simulink library "dinr"  (Simulink 8.2)
settings: Solver=ode45  SolverMode=SingleTasking  StartTime=0.0  StopTime=10.0  RelTol=1e-3
undefined symbols (not defined in the file or in its folder): FALSE, KDINR_DisableEstimator_flg, TRUE
libraries: simulink x2
(part 2 of 2)

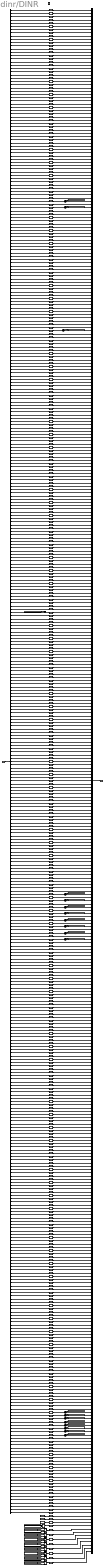
== system dinr/DINR ==
  BINP_outputs : Inport  OutDataTypeStr=Bus: BINP_outputs
  trig_DINR : TriggerPort  TriggerType=function-call
  Bus Selector : BusSelector  OutputSignals=VINP_IgnitionVolt_V,VINP_IgnitionVoltValid_flg,VINP_BatteryVolt_V,VINP_BatteryVoltValid_flg,VINP_AppTime_ms,VINP_ADCFault_enum,VINP_EEPROMFault_enum,VINP_RAMFault_enum,VINP_ROMFault_enum,VINP_VREF1Fault_enum,VINP_VREF2Fault_enum,VINP_AccelPedalPosn_pct,VINP_AccelPedalPosnValid_flg,VINP_EffAccelPedalPosn_pct,VINP_EffAccelPedalPosnValid_flg,VINP_EngSpd_erpm,VINP_EngSpdValid_flg,VINP_EngTqFriction_Nm,VINP_EngTqFrictionValid_flg,VINP_EngTqIndicated_Nm,VINP_EngTqIndicatedValid_flg,VINP_EngTqIndicatedCOR_Nm,VINP_EngTqIndicatedCORValid_flg,VINP_EngTqMax_Nm,VINP_EngTqMaxValid_flg,VINP_EngTqMin_Nm,VINP_EngTqMinValid_flg,VINP_EngTqUnCORFault_flg,VINP_EngTqUnCORFaultValid_flg,VINP_EMSHybridOpState_enum,VINP_EMSHybridOpStateValid_flg,VINP_EMSOpState_enum,VINP_EMSOpStateValid_flg,VINP_EngHoodOpen_flg,VINP_EngHoodOpenValid_flg,VINP_OBDWarnCycAchiv_flg,VINP_OBDWarnCycAchivValid_flg,VINP_OBDDriveCycAchiv_flg,VINP_OBDDriveCycAchivValid_flg,VINP_ShifterPosn_enum,VINP_ShifterPosnValid_flg,VINP_NowGearPosn_enum,VINP_NowGearPosnValid_flg,VINP_TMTurbineSpd_rpm,VINP_TMTurbineSpdValid_flg,VINP_TCMFaultStatus_enum,VINP_TCMFaultStatusValid_flg,VINP_TqConvClutchSt_enum,VINP_TqConvClutchStValid_flg,VINP_TCMMILReq_flg,VINP_TCMMILReqValid_flg,VINP_TCMWinterMode_flg,VINP_TCMWinterModeValid_flg,VINP_TCMPowerMode_flg,VINP_TCMPowerModeValid_flg,VINP_DriverMode_enum,VINP_DriverModeValid_flg,VINP_KeySwitchStatus_enum,VINP_KeySwitchStatusValid_flg,VINP_TurnSignalSwL_flg,VINP_TurnSignalSwLValid_flg,VINP_TurnSignalSwR_flg,VINP_TurnSignalSwRValid_flg,VINP_HazardLightSw_flg,VINP_HazardLightSwValid_flg,VINP_DriverDoorOpen_flg,VINP_DriverDoorOpenValid_flg,VINP_PassengerDoorOpen_flg,VINP_PassengerDoorOpenValid_flg,VINP_LRDoorOpen_flg,VINP_LRDoorOpenValid_flg,VINP_RRDoorOpen_flg,VINP_RRDoorOpenValid_flg,VINP_TailGateOpen_flg,VINP_TailGateOpenValid_flg,VINP_AnyDoorOpen_flg,VINP_AnyDoorOpenValid_flg,VINP_VehCrashed_flg,VINP_VehCrashedValid_flg,VINP_ABSActive_flg,VINP_ABSActiveValid_flg,VINP_ABSFault_flg,VINP_ABSFaultValid_flg,VINP_EBDFault_flg,VINP_EBDFaultValid_flg,VINP_ESCActive_flg,VINP_ESCActiveValid_flg,VINP_ESCFault_flg,VINP_ESCFaultValid_flg,VINP_TCSActive_flg,VINP_TCSActiveValid_flg,VINP_TCSEnabled_flg,VINP_TCSEnabledValid_flg,VINP_TCSFault_flg,VINP_TCSFaultValid_flg,VINP_HSAActive_flg,VINP_HSAActiveValid_flg,VINP_HSAFault_flg,VINP_HSAFaultValid_flg,VINP_BrkLampOn_flg,VINP_BrkLampOnValid_flg,VINP_VehSpd_kph,VINP_VehSpdValid_flg,VINP_YawRate_degps,VINP_YawRateValid_flg,VINP_LatAccel_G,VINP_LatAccelValid_flg,VINP_LongAccel_G,VINP_LongAccelValid_flg,VINP_MCPressure_bar,VINP_MCPressureValid_flg,VINP_SurfaceGrade_deg,VINP_SurfaceGradeValid_flg,VINP_BrakBoosterPres_kPa,VINP_BrakBoosterPresValid_flg,VINP_LowBrakBoosterPres_flg,VINP_LowBrakBoosterPresValid_flg,VINP_LFWheelSpeed_kph,VINP_LFWheelSpeedValid_flg,VINP_LRWheelSpeed_kph,VINP_LRWheelSpeedValid_flg,VINP_RFWheelSpeed_kph,VINP_RFWheelSpeedValid_flg,VINP_RRWheelSpeed_kph,VINP_RRWheelSpeedValid_flg,VINP_SteerAngle_deg,VINP_SteerAngleValid_flg,VINP_SteerSpeed_degps,VINP_SteerSpeedValid_flg,VINP_RelSteerAngle_deg,VINP_RelSteerAngleValid_flg,VINP_SteerTorque_Nm,VINP_SteerTorqueValid_flg,VINP_EPSElectPWR_A,VINP_EPSElectPWRValid_flg,VINP_EPSFailed_flg,VINP_EPSFailedValid_flg,VINP_AckCurStrAngReq_deg,VINP_AckCurStrAngReqValid_flg,VINP_AckCurStrAngReqApplable_flg,VINP_AckCurStrAngReqApplableValid_flg,VINP_AckCurStrTqReq_Nm,VINP_AckCurStrTqReqValid_flg,VINP_AckCurStrTqReqApplable_flg,VINP_AckCurStrTqReqApplableValid_flg,VINP_EPSBattVolt_V,VINP_EPSBattVoltValid_flg,VINP_EPASMILReq_flg,VINP_EPASMILReqValid_flg,VINP_EPSLKAStatus_enum,VINP_EPSLKAStatusValid_flg,VINP_EPSLFCStatus_enum,VINP_EPSLFCStatusValid_flg,VINP_EPSADASAbReason_enum,VINP_EPSADASAbReasonValid_flg,VINP_OdoMeter_km,VINP_OdoMeterValid_flg,VINP_LowBrakeFluid_flg,VINP_LowBrakeFluidValid_flg,VINP_ParkBrakeOn_flg,VINP_ParkBrakeOnValid_flg,VINP_SeatBeltNOTFasten_flg,VINP_SeatBeltNOTFastenValid_flg,VINP_MeterVehSpd_kph,VINP_MeterVehSpdValid_flg,VINP_OutsideTemp_degC,VINP_OutsideTempValid_flg,VINP_ParkBrakeBindSta_enum,VINP_ParkBrakeBindStaValid_flg,VINP_RearFogSwOn_flg,VINP_RearFogSwOnValid_flg,VINP_HighBeamSwOn_flg,VINP_HighBeamSwOnValid_flg,VINP_AckCurBrakDecReq_mps2,VINP_AckCurBrakDecReqValid_flg,VINP_AckCurBrakDecReqApplable_flg,VINP_AckCurBrakDecReqApplableValid_flg,VINP_AckCurPTTqReq_Nm,VINP_AckCurPTTqReqValid_flg,VINP_AckCurPTTqReqApplable_flg,VINP_AckCurPTTqReqApplableValid_flg,VINP_AckCurVehDec_mps2,VINP_AckCurVehDecValid_flg,VINP_DeceContManag_flg,VINP_DeceContManagValid_flg,VINP_DriverBrakPedalOn_flg,VINP_DriverBrakPedalOnValid_flg,VINP_ECMExtnTqAvailable_flg,VINP_ECMExtnTqAvailableValid_flg,VINP_ECMTqSource_enum,VINP_ECMTqSourceValid_flg,VINP_ESCBrakeStatus_enum,VINP_ESCBrakeStatusValid_flg,VINP_ESCExtnBrkAvailable_flg,VINP_ESCExtnBrkAvailableValid_flg,VINP_ESCBattVolt_V,VINP_ESCBattVoltValid_flg,VINP_HWAccelPedalPosn_pct,VINP_HWAccelPedalPosnValid_flg,VINP_CurDriverTqReq_Nm,VINP_CurDriverTqReqValid_flg,VINP_TCMGearPosnReqAllow_enum,VINP_TCMGearPosnReqAllowValid_flg,VINP_MSAStatus_enum,VINP_MSAStatusValid_flg,VINP_HybridLimpHome_flg,VINP_HybridLimpHomeValid_flg,VINP_HCUMILReq_flg,VINP_HCUMILReqValid_flg,VINP_ACCOnVCU_flg,VINP_ACCOnVCUValid_flg,VINP_ACCResSpdIncVCU_flg,VINP_ACCResSpdIncVCUValid_flg,VINP_ACCSetSpdDecVCU_flg,VINP_ACCSetSpdDecVCUValid_flg,VINP_ACCDistVCU_flg,VINP_ACCDistVCUValid_flg,VINP_ACCTimeGapIncVCU_flg,VINP_ACCTimeGapIncVCUValid_flg,VINP_ACCTimeGapDecVCU_flg,VINP_ACCTimeGapDecVCUValid_flg,VINP_LFCOnVCU_flg,VINP_LFCOnVCUValid_flg,VINP_MSAOnVCU_flg,VINP_MSAOnVCUValid_flg,VINP_AEBEnableH_flg,VINP_AEBEnableHValid_flg,VINP_FCWEnableH_flg,VINP_FCWEnableHValid_flg,VINP_CSCEnableH_flg,VINP_CSCEnableHValid_flg,VINP_LKAEnableH_flg,VINP_LKAEnableHValid_flg,VINP_MAPAEnableH_flg,VINP_MAPAEnableHValid_flg,VINP_LCSEnableH_flg,VINP_LCSEnableHValid_flg,VINP_FCWWarningModeH_enum,VINP_FCWWarningModeHValid_flg,VINP_DefMaxACCSetSpeed_kph,VINP_DefMaxACCSetSpeedValid_flg,VINP_LFCPilotOnH_flg,VINP_LFCPilotOnHValid_flg,VINP_LFCPilotCancelH_flg,VINP_LFCPilotCancelHValid_flg,VINP_ACCOnH_flg,VINP_ACCOnHValid_flg,VINP_ACCCancelH_flg,VINP_ACCCancelHValid_flg,VINP_ACCResSpdIncH_flg,VINP_ACCResSpdIncHValid_flg,VINP_ACCSetSpdDecH_flg,VINP_ACCSetSpdDecHValid_flg,VINP_ACCSpdIncH_flg,VINP_ACCSpdIncHValid_flg,VINP_ACCSpdDecH_flg,VINP_ACCSpdDecHValid_flg,VINP_ACCTimeGapIncH_flg,VINP_ACCTimeGapIncHValid_flg,VINP_ACCTimeGapDecH_flg,VINP_ACCTimeGapDecHValid_flg,VINP_IGSAOnH_flg,VINP_IGSAOnHValid_flg,VINP_IGSAResSpdIncH_flg,VINP_IGSAResSpdIncHValid_flg,VINP_IGSASetSpdDecH_flg,VINP_IGSASetSpdDecHValid_flg,VINP_IGSASwitchModeH_flg,VINP_IGSASwitchModeHValid_flg,VINP_LaneQualityL_enum,VINP_LaneQualityLValid_flg,VINP_LaneQualityR_enum,VINP_LaneQualityRValid_flg,VINP_LaneC0LRaw_m,VINP_LaneC0LValid_flg,VINP_LaneC1LRaw_rad,VINP_LaneC1LValid_flg,VINP_LaneC2LRaw_rat,VINP_LaneC2LValid_flg,VINP_LaneC3LRaw_rat,VINP_LaneC3LValid_flg,VINP_LaneC0RRaw_m,VINP_LaneC0RValid_flg,VINP_LaneC1RRaw_rad,VINP_LaneC1RValid_flg,VINP_LaneC2RRaw_rat,VINP_LaneC2RValid_flg,VINP_LaneC3RRaw_rat,VINP_LaneC3RValid_flg,VINP_LaneTypeL_enum,VINP_LaneTypeLValid_flg,VINP_LaneTypeR_enum,VINP_LaneTypeRValid_flg,VINP_LaneMrkClrL_enum,VINP_LaneMrkClrLValid_flg,VINP_LaneMrkClrR_enum,VINP_LaneMrkClrRValid_flg,VINP_LaneMrkWidL_m,VINP_LaneMrkWidLValid_flg,VINP_LaneMrkWidR_m,VINP_LaneMrkWidRValid_flg,VINP_ViewRangeStartL_m,VINP_ViewRangeStartLValid_flg,VINP_ViewRangeStartR_m,VINP_ViewRangeStartRValid_flg,VINP_ViewRangeEndL_m,VINP_ViewRangeEndLValid_flg,VINP_ViewRangeEndR_m,VINP_ViewRangeEndRValid_flg,VINP_TLCL_s,VINP_TLCLValid_flg,VINP_TLCR_s,VINP_TLCRValid_flg,VINP_LaneCrosL_flg,VINP_LaneCrosLValid_flg,VINP_LaneCrosR_flg,VINP_LaneCrosRValid_flg,VINP_NextLaneC0L_m,VINP_NextLaneC0LValid_flg,VINP_NextLaneC1L_rad,VINP_NextLaneC1LValid_flg,VINP_NextLaneC2L_rat,VINP_NextLaneC2LValid_flg,VINP_NextLaneC3L_rat,VINP_NextLaneC3LValid_flg,VINP_NextLaneQualityL_enum,VINP_NextLaneQualityLValid_flg,VINP_NextLaneTypeL_enum,VINP_NextLaneTypeLValid_flg,VINP_NextLaneMrkWidL_m,VINP_NextLaneMrkWidLValid_flg,VINP_NextViewRangeStartL_m,VINP_NextViewRangeStartLValid_flg,VINP_NextViewRangeEndL_m,VINP_NextViewRangeEndLValid_flg,VINP_NextLaneC0R_m,VINP_NextLaneC0RValid_flg,VINP_NextLaneC1R_rad,VINP_NextLaneC1RValid_flg,VINP_NextLaneC2R_rat,VINP_NextLaneC2RValid_flg,VINP_NextLaneC3R_rat,VINP_NextLaneC3RValid_flg,VINP_NextLaneQualityR_enum,VINP_NextLaneQualityRValid_flg,VINP_NextLaneTypeR_enum,VINP_NextLaneTypeRValid_flg,VINP_NextLaneMrkWidR_m,VINP_NextLaneMrkWidRValid_flg,VINP_NextViewRangeStartR_m,VINP_NextViewRangeStartRValid_flg,VINP_NextViewRangeEndR_m,VINP_NextViewRangeEndRValid_flg,VINP_CamNofObjects_num,VINP_CamNofObjectsValid_flg,VINP_CamGoDecision_enum,VINP_CamGoDecisionValid_flg,VINP_CloseCarDetected_flg,VINP_CloseCarDetectedValid_flg,VINP_RightCarCutIn_flg,VINP_RightCarCutInValid_flg,VINP_LeftCarCutIn_flg,VINP_LeftCarCutInValid_flg,VINP_CamFSImpairedVD_flg,VINP_CamFSImpairedVDValid_flg,VINP_CamFSLowSun_flg,VINP_CamFSLowSunValid_flg,VINP_CamFSBlurImage_flg,VINP_CamFSBlurImageValid_flg,VINP_CamFSSmearImage_flg,VINP_CamFSSmearImageValid_flg,VINP_CamFSPartialBlockage_flg,VINP_CamFSPartialBlockageValid_flg,VINP_CamFSFullBlockage_flg,VINP_CamFSFullBlockageValid_flg,VINP_CamFSSplashes_flg,VINP_CamFSSplashesValid_flg,VINP_CamFSOutofCal_flg,VINP_CamFSOutofCalValid_flg,VINP_CamFSCalMisalign_flg,VINP_CamFSCalMisalignValid_flg,VINP_CamFSSmearedspots_flg,VINP_CamFSSmearedspotsValid_flg,VINP_CamFSSpotHalosFrozen_flg,VINP_CamFSSpotHalosFrozenValid_flg,VINP_CamFSFoggySpots_flg,VINP_CamFSFoggySpotsValid_flg,VINP_CamFSSunRay_flg,VINP_CamFSSunRayValid_flg,VINP_CamObsID10_num,VINP_CamObsIDValid10_flg,VINP_CamObsPosX10_m,VINP_CamObsPosXValid10_flg,VINP_CamObsPosY10_m,VINP_CamObsPosYValid10_flg,VINP_CamObsVelX10_mps,VINP_CamObsVelXValid10_flg,VINP_CamObsVelY10_mps,VINP_CamObsVelYValid10_flg,VINP_CamObsAccX10_mps2,VINP_CamObsAccXValid10_flg,VINP_CamObsAng10_deg,VINP_CamObsAngValid10_flg,VINP_CamObsAngRate10_degps,VINP_CamObsAngRateValid10_flg,VINP_CamObsLength10_m,VINP_CamObsLengthValid10_flg,VINP_CamObsWidth10_m,VINP_CamObsWidthValid10_flg,VINP_CamObsType10_enum,VINP_CamObsTypeValid10_flg,VINP_CamObsStatus10_enum,VINP_CamObsStatusValid10_flg,VINP_CamObsValid10_enum,VINP_CamObsValidValid10_flg,VINP_CamObsMoveInO10_enum,VINP_CamObsMoveInOValid10_flg,VINP_CamObsBlinker10_enum,VINP_CamObsBlinkerValid10_flg,VINP_CamObsBrakeLight10_flg,VINP_CamObsBrakeLightValid10_flg,VINP_CamObsAge10_cnt,VINP_CamObsAgeValid10_flg,VINP_CamObsLane10_enum,VINP_CamObsLaneValid10_flg,VINP_CamObsCIPV10_flg,VINP_CamObsCIPVValid10_flg,VINP_CamObsReplaced10_flg,VINP_CamObsReplacedValid10_flg,VINP_IgnitionActive_flg,VINP_VehSpd_mps,VINP_SteerAngle_rad,VINP_YawRate_radps,VINP_LaneC0LKalF_m,VINP_LaneC1LKalF_rad,VINP_LaneC2LKalF_rat,VINP_LaneC3LKalF_rat,VINP_LaneC0RKalF_m,VINP_LaneC1RKalF_rad,VINP_LaneC2RKalF_rat,VINP_LaneC3RKalF_rat,VINP_ABSCANValid_flg,VINP_BCMCANValid_flg,VINP_ECMCANValid_flg,VINP_TCMCANValid_flg,VINP_EPSCANValid_flg,VINP_METERCANValid_flg,VINP_ACCANValid_flg,VINP_EPBCANValid_flg,VINP_VCUCANValid_flg,VINP_HMICANValid_flg,VINP_CSWCANValid_flg,VINP_EPMCANValid_flg,VINP_ABSCANAlive_flg,VINP_BCMCANAlive_flg,VINP_ECMCANAlive_flg,VINP_TCMCANAlive_flg,VINP_EPSCANAlive_flg,VINP_METERCANAlive_flg,VINP_ACCANAlive_flg,VINP_EPBCANAlive_flg,VINP_VCUCANAlive_flg,VINP_HMICANAlive_flg,VINP_CSWCANAlive_flg,VINP_EPMCANAlive_flg
  Bus1 : BusCreator  Inputs=477  OutDataTypeStr=Bus: BDINR_outputs
  Cast{1,3,5,7,9,11,13,15,17,19,21,23,25,27,29,31..33,35,37..43,46..47,49,51,53,55,57,59,61,64..65,67,69,71,73,75,77,79,184,224..225,341,354..357,360,363,365,367,369,371,374,376,378,380..385,387,389,391,393,395..396,398,400..401,403,405..406,408..410,412..414,416..419,422,424..425,427..434,436,439..440,442..445,448,450..454,456,458..460,462..464,466,468,470,472..486,489..498,500..502,504..505,507,509,511..518,520,522..524,526,529,531..533,535,537,539..560,562..572,574..583,585..591,593..605,607,609,611..613,615,617..620,622..627,629..649,651..671,673..674,676,679,684,691..705,715..716,718..726,729..731,733..738} (335 alike) : DataTypeConversion  OutDataTypeStr=boolean  RndMeth=Zero
  Cast{4,6,8,10,12,14,16,18,20,44..45,48,50,56,58,60,62..63,66,68,74,76,78,342..349,368,370,372,375,377,379,386,388,390,392,394,399,402,404,407,411,415,420,426,435,437,446..447,449,461,467,487..488,499,503,506,508,525,527..528,534,536,561,584,606,608,610,614,621,628,650,672,675,677..678,682..683,685..690,706..714,727} (99 alike) : DataTypeConversion  OutDataTypeStr=single  RndMeth=Zero
  Cast{2,22,24,26,28,30,34,36,52,54,70,72,185,358..359,361..362,364,366,373,397,421,423,438,441,455,457,465,469,471,510,519,521,530,538,573,592,616,680..681,717,728,732} (43 alike) : DataTypeConversion  OutDataTypeStr=uint8  RndMeth=Zero
  Constant : Constant  Value=FALSE
  Constant1 : Constant  Value=TRUE
  Constant2 : Constant  Value=TRUE
  Logical Operator : Logic  Operator=OR  AllPortsSameDT=off  OutDataTypeStr=boolean
  Switch{1..6,8..9} (8 alike) : Switch  Criteria=u2 ~= 0
  Terminator : Terminator
  ovrdflg{1..5,7..9} (8 alike) : Constant  Value=KDINR_DisableEstimator_flg
  BDINR_outputs : Outport  OutDataTypeStr=Bus: BDINR_outputs
  wires:
  Logical Operator/1 -> Cast341/1
  Cast341/1 -> Bus1/469  "VDINR_TurnSignalSw_flg"
  Cast342/1 -> Bus1/470  "VDINR_LaneC0L_m"
  Switch8/1 -> Cast342/1
  ovrdflg8/1 -> Switch8/2
  BINP_outputs/1 -> Bus Selector/1
  [VDINR_TurnSignalSwL_flg] -> Logical Operator/1
  [VDINR_TurnSignalSwR_flg] -> Logical Operator/2
  [VDINR_LaneC0LRaw_m] -> Switch8/1
  [VDINR_LaneC0LKalF_m] -> Switch8/3
  Cast343/1 -> Bus1/471  "VDINR_LaneC1L_rad"
  Switch9/1 -> Cast343/1
  ovrdflg9/1 -> Switch9/2
  [VDINR_LaneC1LRaw_rad] -> Switch9/1
  [VDINR_LaneC1LKalF_rad] -> Switch9/3
  Cast344/1 -> Bus1/472  "VDINR_LaneC2L_rat"
  Switch1/1 -> Cast344/1
  ovrdflg1/1 -> Switch1/2
  [VDINR_LaneC2LKalF_rat] -> Switch1/3
  [VDINR_LaneC2LRaw_rat] -> Switch1/1
  Cast345/1 -> Bus1/473  "VDINR_LaneC3L_rat"
  Switch2/1 -> Cast345/1
  ovrdflg2/1 -> Switch2/2
  [VDINR_LaneC3LKalF_rat] -> Switch2/3
  [VDINR_LaneC3LRaw_rat] -> Switch2/1
  Cast346/1 -> Bus1/474  "VDINR_LaneC0R_m"
  Switch3/1 -> Cast346/1
  ovrdflg3/1 -> Switch3/2
  [VDINR_LaneC0RKalF_m] -> Switch3/3
  [VDINR_LaneC0RRaw_m] -> Switch3/1
  Cast347/1 -> Bus1/475  "VDINR_LaneC1R_rad"
  Switch4/1 -> Cast347/1
  ovrdflg7/1 -> Switch4/2
  [VDINR_LaneC1RKalF_rad] -> Switch4/3
  [VDINR_LaneC1RRaw_rad] -> Switch4/1
  Cast348/1 -> Bus1/476  "VDINR_LaneC2R_rat"
  Switch5/1 -> Cast348/1
  ovrdflg4/1 -> Switch5/2
  [VDINR_LaneC2RKalF_rat] -> Switch5/3
  [VDINR_LaneC2RRaw_rat] -> Switch5/1
  Cast349/1 -> Bus1/477  "VDINR_LaneC3R_rat"
  Switch6/1 -> Cast349/1
  ovrdflg5/1 -> Switch6/2
  [VDINR_LaneC3RKalF_rat] -> Switch6/3
  [VDINR_LaneC3RRaw_rat] -> Switch6/1
  Bus1/1 -> BDINR_outputs/1  "BDINR_outputs"
  Cast461/1 -> Bus1/1  "VDINR_IgnitionVolt_V"
  Cast572/1 -> Bus1/2  "VDINR_IgnitionVoltValid_flg"
  Cast695/1 -> Bus1/430  "VDINR_IgnitionActive_flg"
  Cast706/1 -> Bus1/5  "VDINR_AppTime_ms"
  Cast561/1 -> Bus1/431  "VDINR_VehSpd_mps"
  Cast584/1 -> Bus1/432  "VDINR_SteerAngle_rad"
  Cast606/1 -> Bus1/433  "VDINR_YawRate_radps"
  Cast680/1 -> Bus1/270  "VDINR_LaneQualityL_enum"
  Cast681/1 -> Bus1/272  "VDINR_LaneQualityR_enum"
  Cast362/1 -> Bus1/10  "VDINR_VREF1Fault_enum"
  Cast373/1 -> Bus1/11  "VDINR_VREF2Fault_enum"
  Cast717/1 -> Bus1/7  "VDINR_EEPROMFault_enum"
  Cast728/1 -> Bus1/8  "VDINR_RAMFault_enum"
  Cast185/1 -> Bus1/9  "VDINR_ROMFault_enum"
  Cast735/1 -> Bus1/271  "VDINR_LaneQualityLValid_flg"
  Cast736/1 -> Bus1/273  "VDINR_LaneQualityRValid_flg"
  Cast737/1 -> Bus1/275  "VDINR_LaneC0LValid_flg"
  Cast738/1 -> Bus1/277  "VDINR_LaneC1LValid_flg"
  Cast224/1 -> Bus1/279  "VDINR_LaneC2LValid_flg"
  Cast225/1 -> Bus1/281  "VDINR_LaneC3LValid_flg"
  Cast354/1 -> Bus1/283  "VDINR_LaneC0RValid_flg"
  Cast355/1 -> Bus1/285  "VDINR_LaneC1RValid_flg"
  Cast356/1 -> Bus1/287  "VDINR_LaneC2RValid_flg"
  Cast357/1 -> Bus1/289  "VDINR_LaneC3RValid_flg"
  Cast358/1 -> Bus1/6  "VDINR_ADCFault_enum"
  Cast359/1 -> Bus1/290  "VDINR_LaneTypeL_enum"
  Cast360/1 -> Bus1/291  "VDINR_LaneTypeLValid_flg"
  Cast361/1 -> Bus1/292  "VDINR_LaneTypeR_enum"
  Cast363/1 -> Bus1/293  "VDINR_LaneTypeRValid_flg"
  Cast364/1 -> Bus1/294  "VDINR_LaneMrkClrL_enum"
  Cast365/1 -> Bus1/295  "VDINR_LaneMrkClrLValid_flg"
  Cast366/1 -> Bus1/296  "VDINR_LaneMrkClrR_enum"
  Cast367/1 -> Bus1/297  "VDINR_LaneMrkClrRValid_flg"
  Cast368/1 -> Bus1/298  "VDINR_LaneMrkWidL_m"
  Cast369/1 -> Bus1/299  "VDINR_LaneMrkWidLValid_flg"
  Cast370/1 -> Bus1/300  "VDINR_LaneMrkWidR_m"
  Cast371/1 -> Bus1/301  "VDINR_LaneMrkWidRValid_flg"
  Cast372/1 -> Bus1/302  "VDINR_ViewRangeStartL_m"
  Cast374/1 -> Bus1/303  "VDINR_ViewRangeStartLValid_flg"
  Cast375/1 -> Bus1/304  "VDINR_ViewRangeStartR_m"
  Cast376/1 -> Bus1/305  "VDINR_ViewRangeStartRValid_flg"
  Cast377/1 -> Bus1/310  "VDINR_TLCL_s"
  Cast378/1 -> Bus1/311  "VDINR_TLCLValid_flg"
  Cast379/1 -> Bus1/312  "VDINR_TLCR_s"
  Cast380/1 -> Bus1/313  "VDINR_TLCRValid_flg"
  Cast381/1 -> Bus1/314  "VDINR_LaneCrosL_flg"
  Cast382/1 -> Bus1/315  "VDINR_LaneCrosLValid_flg"
  Cast383/1 -> Bus1/316  "VDINR_LaneCrosR_flg"
  Cast385/1 -> Bus1/317  "VDINR_LaneCrosRValid_flg"
  Cast677/1 -> Bus1/12  "VDINR_AccelPedalPosn_pct"
  Cast679/1 -> Bus1/13  "VDINR_AccelPedalPosnValid_flg"
  Cast716/1 -> Bus1/80  "VDINR_ABSActive_flg"
  Cast718/1 -> Bus1/82  "VDINR_ABSFault_flg"
  Cast719/1 -> Bus1/100, [VDINR_BrkLampOn_flg]  "VDINR_BrkLampOn_flg"
  Cast720/1 -> Bus1/101  "VDINR_BrkLampOnValid_flg"
  Cast721/1 -> Bus1/84  "VDINR_EBDFault_flg"
  Cast722/1 -> Bus1/86  "VDINR_ESCActive_flg"
  Cast723/1 -> Bus1/88  "VDINR_ESCFault_flg"
  Cast724/1 -> Bus1/90  "VDINR_TCSActive_flg"
  Cast725/1 -> Bus1/92  "VDINR_TCSEnabled_flg"
  Cast726/1 -> Bus1/94  "VDINR_TCSFault_flg"
  Cast727/1 -> Bus1/102  "VDINR_VehSpd_kph"
  Cast729/1 -> Bus1/103  "VDINR_VehSpdValid_flg"
  Cast730/1 -> Bus1/127  "VDINR_SteerAngleValid_flg"
  Cast731/1 -> Bus1/105  "VDINR_YawRateValid_flg"
  Cast732/1 -> Bus1/58  "VDINR_KeySwitchStatus_enum"
  Cast441/1 -> Bus1/40  "VDINR_ShifterPosn_enum"
  Cast443/1 -> Bus1/41  "VDINR_ShifterPosnValid_flg"
  Cast446/1 -> Bus1/134  "VDINR_EPSElectPWR_A"
  Cast453/1 -> Bus1/59  "VDINR_KeySwitchStatusValid_flg"
  Cast475/1 -> Bus1/61  "VDINR_TurnSignalSwLValid_flg"
  Cast476/1 -> Bus1/63  "VDINR_TurnSignalSwRValid_flg"
  Cast478/1 -> Bus1/81  "VDINR_ABSActiveValid_flg"
  Cast479/1 -> Bus1/83  "VDINR_ABSFaultValid_flg"
  Cast480/1 -> Bus1/85  "VDINR_EBDFaultValid_flg"
  Cast481/1 -> Bus1/87  "VDINR_ESCActiveValid_flg"
  Cast482/1 -> Bus1/89  "VDINR_ESCFaultValid_flg"
  Cast483/1 -> Bus1/91  "VDINR_TCSActiveValid_flg"
  Cast485/1 -> Bus1/93  "VDINR_TCSEnabledValid_flg"
  Cast486/1 -> Bus1/95  "VDINR_TCSFaultValid_flg"
  Cast487/1 -> Bus1/126  "VDINR_SteerAngle_deg"
  Cast488/1 -> Bus1/104  "VDINR_YawRate_degps"
  Cast491/1 -> Bus1/135  "VDINR_EPSElectPWRValid_flg"
  Cast386/1 -> Bus1/14  "VDINR_EffAccelPedalPosn_pct"
  Cast387/1 -> Bus1/15  "VDINR_EffAccelPedalPosnValid_flg"
  Cast388/1 -> Bus1/16  "VDINR_EngSpd_erpm"
  Cast389/1 -> Bus1/17  "VDINR_EngSpdValid_flg"
  Cast390/1 -> Bus1/18  "VDINR_EngTqFriction_Nm"
  Cast391/1 -> Bus1/19  "VDINR_EngTqFrictionValid_flg"
  Cast392/1 -> Bus1/24  "VDINR_EngTqMax_Nm"
  Cast393/1 -> Bus1/25  "VDINR_EngTqMaxValid_flg"
  Cast394/1 -> Bus1/26  "VDINR_EngTqMin_Nm"
  Cast396/1 -> Bus1/27  "VDINR_EngTqMinValid_flg"
  Cast399/1 -> Bus1/132  "VDINR_SteerTorque_Nm"
  Cast400/1 -> Bus1/133  "VDINR_SteerTorqueValid_flg"
  Cast401/1 -> Bus1/107  "VDINR_LatAccelValid_flg"
  Cast402/1 -> Bus1/106  "VDINR_LatAccel_G"
  Cast403/1 -> Bus1/109  "VDINR_LongAccelValid_flg"
  Cast404/1 -> Bus1/108  "VDINR_LongAccel_G"
  Cast405/1 -> Bus1/111  "VDINR_MCPressureValid_flg"
  Cast407/1 -> Bus1/110  "VDINR_MCPressure_bar"
  Cast447/1 -> Bus1/20  "VDINR_EngTqIndicated_Nm"
  Cast448/1 -> Bus1/21  "VDINR_EngTqIndicatedValid_flg"
  Cast449/1 -> Bus1/22  "VDINR_EngTqIndicatedCOR_Nm"
  Cast451/1 -> Bus1/23  "VDINR_EngTqIndicatedCORValid_flg"
  Cast452/1 -> Bus1/28  "VDINR_EngTqUnCORFault_flg"
  Cast454/1 -> Bus1/29  "VDINR_EngTqUnCORFaultValid_flg"
  Cast455/1 -> Bus1/30  "VDINR_EMSHybridOpState_enum"
  Cast456/1 -> Bus1/31  "VDINR_EMSHybridOpStateValid_flg"
  Cast457/1 -> Bus1/32  "VDINR_EMSOpState_enum"
  Cast458/1 -> Bus1/33  "VDINR_EMSOpStateValid_flg"
  Cast459/1 -> Bus1/34  "VDINR_EngHoodOpen_flg"
  Cast460/1 -> Bus1/35  "VDINR_EngHoodOpenValid_flg"
  Cast465/1 -> Bus1/42  "VDINR_NowGearPosn_enum"
  Cast466/1 -> Bus1/43  "VDINR_NowGearPosnValid_flg"
  Cast467/1 -> Bus1/44  "VDINR_TMTurbineSpd_rpm"
  Cast468/1 -> Bus1/45  "VDINR_TMTurbineSpdValid_flg"
  Cast469/1 -> Bus1/46  "VDINR_TCMFaultStatus_enum"
  Cast470/1 -> Bus1/47  "VDINR_TCMFaultStatusValid_flg"
  Cast471/1 -> Bus1/56  "VDINR_DriverMode_enum"
  Cast472/1 -> Bus1/57  "VDINR_DriverModeValid_flg"
  Cast474/1 -> Bus1/64  "VDINR_HazardLightSw_flg"
  Cast477/1 -> Bus1/65  "VDINR_HazardLightSwValid_flg"
  Cast492/1 -> Bus1/66  "VDINR_DriverDoorOpen_flg"
  Cast493/1 -> Bus1/67  "VDINR_DriverDoorOpenValid_flg"
  Cast494/1 -> Bus1/68  "VDINR_PassengerDoorOpen_flg"
  Cast496/1 -> Bus1/69  "VDINR_PassengerDoorOpenValid_flg"
  Cast497/1 -> Bus1/70  "VDINR_LRDoorOpen_flg"
  Cast498/1 -> Bus1/71  "VDINR_LRDoorOpenValid_flg"
  Cast673/1 -> Bus1/72  "VDINR_RRDoorOpen_flg"
  Cast684/1 -> Bus1/73  "VDINR_RRDoorOpenValid_flg"
  Cast384/1 -> Bus1/74  "VDINR_TailGateOpen_flg"
  Cast395/1 -> Bus1/75  "VDINR_TailGateOpenValid_flg"
  Cast406/1 -> Bus1/76  "VDINR_AnyDoorOpen_flg"
  Cast417/1 -> Bus1/77  "VDINR_AnyDoorOpenValid_flg"
  Cast428/1 -> Bus1/78  "VDINR_VehCrashed_flg"
  Cast439/1 -> Bus1/79  "VDINR_VehCrashedValid_flg"
  Cast450/1 -> Bus1/96  "VDINR_HSAActive_flg"
  Cast462/1 -> Bus1/97  "VDINR_HSAActiveValid_flg"
  Cast473/1 -> Bus1/98  "VDINR_HSAFault_flg"
  Cast484/1 -> Bus1/99  "VDINR_HSAFaultValid_flg"
  Cast495/1 -> Bus1/113  "VDINR_SurfaceGradeValid_flg"
  Cast506/1 -> Bus1/112  "VDINR_SurfaceGrade_deg"
  Cast517/1 -> Bus1/115  "VDINR_BrakBoosterPresValid_flg"
  Cast528/1 -> Bus1/114  "VDINR_BrakBoosterPres_kPa"
  Cast539/1 -> Bus1/116  "VDINR_LowBrakBoosterPres_flg"
  Cast550/1 -> Bus1/117  "VDINR_LowBrakBoosterPresValid_flg"
  Cast617/1 -> Bus1/119  "VDINR_LFWheelSpeedValid_flg"
  Cast628/1 -> Bus1/118  "VDINR_LFWheelSpeed_kph"
  Cast639/1 -> Bus1/121  "VDINR_LRWheelSpeedValid_flg"
  Cast650/1 -> Bus1/120  "VDINR_LRWheelSpeed_kph"
  Cast661/1 -> Bus1/123  "VDINR_RFWheelSpeedValid_flg"
  Cast672/1 -> Bus1/122  "VDINR_RFWheelSpeed_kph"
  Cast674/1 -> Bus1/125  "VDINR_RRWheelSpeedValid_flg"
  Cast675/1 -> Bus1/124  "VDINR_RRWheelSpeed_kph"
  Cast676/1 -> Bus1/131  "VDINR_RelSteerAngleValid_flg"
  Cast678/1 -> Bus1/130  "VDINR_RelSteerAngle_deg"
  Cast408/1 -> Bus1/136  "VDINR_EPSFailed_flg"
  Cast409/1 -> Bus1/137  "VDINR_EPSFailedValid_flg"
  Cast410/1 -> Bus1/139  "VDINR_AckCurStrAngReqValid_flg"
  Cast411/1 -> Bus1/138  "VDINR_AckCurStrAngReq_deg"
  Cast412/1 -> Bus1/140  "VDINR_AckCurStrAngReqApplable_flg"
  Cast413/1 -> Bus1/141  "VDINR_AckCurStrAngReqApplableValid_flg"
  Cast414/1 -> Bus1/143  "VDINR_AckCurStrTqReqValid_flg"
  Cast415/1 -> Bus1/142  "VDINR_AckCurStrTqReq_Nm"
  Cast416/1 -> Bus1/144  "VDINR_AckCurStrTqReqApplable_flg"
  Cast418/1 -> Bus1/145  "VDINR_AckCurStrTqReqApplableValid_flg"
  Cast419/1 -> Bus1/147  "VDINR_EPSBattVoltValid_flg"
  Cast420/1 -> Bus1/146  "VDINR_EPSBattVolt_V"
  Cast425/1 -> Bus1/157  "VDINR_OdoMeterValid_flg"
  Cast426/1 -> Bus1/156  "VDINR_OdoMeter_km"
  Cast427/1 -> Bus1/158  "VDINR_LowBrakeFluid_flg"
  Cast429/1 -> Bus1/159  "VDINR_LowBrakeFluidValid_flg"
  Cast430/1 -> Bus1/160  "VDINR_ParkBrakeOn_flg"
  Cast431/1 -> Bus1/161  "VDINR_ParkBrakeOnValid_flg"
  Cast432/1 -> Bus1/162  "VDINR_SeatBeltNOTFasten_flg"
  Cast433/1 -> Bus1/163  "VDINR_SeatBeltNOTFastenValid_flg"
  Cast434/1 -> Bus1/165  "VDINR_MeterVehSpdValid_flg"
  Cast435/1 -> Bus1/164  "VDINR_MeterVehSpd_kph"
  Cast436/1 -> Bus1/167  "VDINR_OutsideTempValid_flg"
  Cast437/1 -> Bus1/166  "VDINR_OutsideTemp_degC"
  Cast438/1 -> Bus1/168  "VDINR_ParkBrakeBindSta_enum"
  Cast440/1 -> Bus1/169  "VDINR_ParkBrakeBindStaValid_flg"
  Cast499/1 -> Bus1/174  "VDINR_AckCurBrakDecReq_mps2"
  Cast500/1 -> Bus1/175  "VDINR_AckCurBrakDecReqValid_flg"
  Cast501/1 -> Bus1/176  "VDINR_AckCurBrakDecReqApplable_flg"
  Cast502/1 -> Bus1/177  "VDINR_AckCurBrakDecReqApplableValid_flg"
  Cast503/1 -> Bus1/178  "VDINR_AckCurPTTqReq_Nm"
  Cast504/1 -> Bus1/179  "VDINR_AckCurPTTqReqValid_flg"
  Cast505/1 -> Bus1/180  "VDINR_AckCurPTTqReqApplable_flg"
  Cast507/1 -> Bus1/181  "VDINR_AckCurPTTqReqApplableValid_flg"
  Cast508/1 -> Bus1/182  "VDINR_AckCurVehDec_mps2"
  Cast509/1 -> Bus1/183  "VDINR_AckCurVehDecValid_flg"
  Cast512/1 -> Bus1/184  "VDINR_DeceContManag_flg"
  Cast513/1 -> Bus1/185  "VDINR_DeceContManagValid_flg"
  Cast514/1 -> Bus1/186  "VDINR_DriverBrakPedalOn_flg"
  Cast515/1 -> Bus1/187  "VDINR_DriverBrakPedalOnValid_flg"
  Cast516/1 -> Bus1/188  "VDINR_ECMExtnTqAvailable_flg"
  Cast518/1 -> Bus1/189  "VDINR_ECMExtnTqAvailableValid_flg"
  Cast519/1 -> Bus1/190  "VDINR_ECMTqSource_enum"
  Cast520/1 -> Bus1/191  "VDINR_ECMTqSourceValid_flg"
  Cast521/1 -> Bus1/192  "VDINR_ESCBrakeStatus_enum"
  Cast522/1 -> Bus1/193  "VDINR_ESCBrakeStatusValid_flg"
  Cast523/1 -> Bus1/194  "VDINR_ESCExtnBrkAvailable_flg"
  Cast524/1 -> Bus1/195  "VDINR_ESCExtnBrkAvailableValid_flg"
  Cast525/1 -> Bus1/196  "VDINR_ESCBattVolt_V"
  Cast526/1 -> Bus1/197  "VDINR_ESCBattVoltValid_flg"
  Cast527/1 -> Bus1/198  "VDINR_HWAccelPedalPosn_pct"
  Cast529/1 -> Bus1/199  "VDINR_HWAccelPedalPosnValid_flg"
  Cast532/1 -> Bus1/208  "VDINR_HCUMILReq_flg"
  Cast533/1 -> Bus1/209  "VDINR_HCUMILReqValid_flg"
  Cast541/1 -> Bus1/218  "VDINR_ACCTimeGapIncVCU_flg"
  Cast542/1 -> Bus1/219  "VDINR_ACCTimeGapIncVCUValid_flg"
  Cast543/1 -> Bus1/220  "VDINR_ACCTimeGapDecVCU_flg"
  Cast544/1 -> Bus1/221  "VDINR_ACCTimeGapDecVCUValid_flg"
  Cast545/1 -> Bus1/222  "VDINR_LFCOnVCU_flg"
  Cast546/1 -> Bus1/223  "VDINR_LFCOnVCUValid_flg"
  Cast547/1 -> Bus1/226  "VDINR_AEBEnableH_flg"
  Cast548/1 -> Bus1/227  "VDINR_AEBEnableHValid_flg"
  Cast549/1 -> Bus1/228  "VDINR_FCWEnableH_flg"
  Cast551/1 -> Bus1/229  "VDINR_FCWEnableHValid_flg"
  Cast552/1 -> Bus1/230  "VDINR_CSCEnableH_flg"
  Cast553/1 -> Bus1/231  "VDINR_CSCEnableHValid_flg"
  Cast554/1 -> Bus1/232  "VDINR_LKAEnableH_flg"
  Cast555/1 -> Bus1/233  "VDINR_LKAEnableHValid_flg"
  Cast556/1 -> Bus1/234  "VDINR_MAPAEnableH_flg"
  Cast557/1 -> Bus1/235  "VDINR_MAPAEnableHValid_flg"
  Cast558/1 -> Bus1/236  "VDINR_LCSEnableH_flg"
  Cast559/1 -> Bus1/237  "VDINR_LCSEnableHValid_flg"
  Cast560/1 -> Bus1/242  "VDINR_LFCPilotOnH_flg"
  Cast562/1 -> Bus1/243  "VDINR_LFCPilotOnHValid_flg"
  Cast563/1 -> Bus1/244  "VDINR_LFCPilotCancelH_flg"
  Cast564/1 -> Bus1/245  "VDINR_LFCPilotCancelHValid_flg"
  Cast565/1 -> Bus1/246  "VDINR_ACCOnH_flg"
  Cast566/1 -> Bus1/247  "VDINR_ACCOnHValid_flg"
  Cast567/1 -> Bus1/248  "VDINR_ACCCancelH_flg"
  Cast568/1 -> Bus1/249  "VDINR_ACCCancelHValid_flg"
  Cast569/1 -> Bus1/250  "VDINR_ACCResSpdIncH_flg"
  Cast570/1 -> Bus1/251  "VDINR_ACCResSpdIncHValid_flg"
  Cast571/1 -> Bus1/252  "VDINR_ACCSetSpdDecH_flg"
  Cast574/1 -> Bus1/253  "VDINR_ACCSetSpdDecHValid_flg"
  Cast575/1 -> Bus1/254  "VDINR_ACCSpdIncH_flg"
  Cast576/1 -> Bus1/255  "VDINR_ACCSpdIncHValid_flg"
  Cast577/1 -> Bus1/256  "VDINR_ACCSpdDecH_flg"
  Cast578/1 -> Bus1/257  "VDINR_ACCSpdDecHValid_flg"
  Cast579/1 -> Bus1/258  "VDINR_ACCTimeGapIncH_flg"
  Cast580/1 -> Bus1/259  "VDINR_ACCTimeGapIncHValid_flg"
  Cast581/1 -> Bus1/260  "VDINR_ACCTimeGapDecH_flg"
  Cast582/1 -> Bus1/261  "VDINR_ACCTimeGapDecHValid_flg"
  Cast583/1 -> Bus1/262  "VDINR_IGSAOnH_flg"
  Cast585/1 -> Bus1/263  "VDINR_IGSAOnHValid_flg"
  Cast586/1 -> Bus1/264  "VDINR_IGSAResSpdIncH_flg"
  Cast587/1 -> Bus1/265  "VDINR_IGSAResSpdIncHValid_flg"
  Cast588/1 -> Bus1/266  "VDINR_IGSASetSpdDecH_flg"
  Cast589/1 -> Bus1/267  "VDINR_IGSASetSpdDecHValid_flg"
  Cast590/1 -> Bus1/268  "VDINR_IGSASwitchModeH_flg"
  Cast591/1 -> Bus1/269  "VDINR_IGSASwitchModeHValid_flg"
  Cast700/1 -> Bus1/442  "VDINR_ABSCANValid_flg"
  Cast701/1 -> Bus1/454  "VDINR_ABSCANAlive_flg"
  Cast704/1 -> Bus1/443  "VDINR_BCMCANValid_flg"
  Cast705/1 -> Bus1/455  "VDINR_BCMCANAlive_flg"
  Cast597/1 -> Bus1/444  "VDINR_ECMCANValid_flg"
  Cast598/1 -> Bus1/456  "VDINR_ECMCANAlive_flg"
  Cast599/1 -> Bus1/445  "VDINR_TCMCANValid_flg"
  Cast600/1 -> Bus1/457  "VDINR_TCMCANAlive_flg"
  Cast601/1 -> Bus1/446  "VDINR_EPSCANValid_flg"
  Cast602/1 -> Bus1/458  "VDINR_EPSCANAlive_flg"
  Cast691/1 -> Bus1/447  "VDINR_METERCANValid_flg"
  Cast692/1 -> Bus1/448  "VDINR_ACCANValid_flg"
  Cast693/1 -> Bus1/449  "VDINR_EPBCANValid_flg"
  Cast694/1 -> Bus1/450  "VDINR_VCUCANValid_flg"
  Cast696/1 -> Bus1/459  "VDINR_METERCANAlive_flg"
  Cast697/1 -> Bus1/460  "VDINR_ACCANAlive_flg"
  Cast698/1 -> Bus1/461  "VDINR_EPBCANAlive_flg"
  Cast699/1 -> Bus1/462  "VDINR_VCUCANAlive_flg"
  Cast603/1 -> Bus1/451  "VDINR_HMICANValid_flg"
  Cast604/1 -> Bus1/453  "VDINR_EPMCANValid_flg"
  Cast605/1 -> Bus1/463  "VDINR_HMICANAlive_flg"
  Cast607/1 -> Bus1/465  "VDINR_EPMCANAlive_flg"
  Cast608/1 -> Bus1/3  "VDINR_BatteryVolt_V"
  Cast609/1 -> Bus1/4  "VDINR_BatteryVoltValid_flg"
  Cast611/1 -> Bus1/129  "VDINR_SteerSpeedValid_flg"
  Cast610/1 -> Bus1/128  "VDINR_SteerSpeed_degps"
  Cast612/1 -> Bus1/148  "VDINR_EPASMILReq_flg"
  Cast613/1 -> Bus1/149  "VDINR_EPASMILReqValid_flg"
  Cast614/1 -> Bus1/200  "VDINR_CurDriverTqReq_Nm"
  Cast615/1 -> Bus1/201  "VDINR_CurDriverTqReqValid_flg"
  Cast616/1 -> Bus1/238  "VDINR_FCWWarningModeH_enum"
  Cast618/1 -> Bus1/239  "VDINR_FCWWarningModeHValid_flg"
  Cast619/1 -> Bus1/224  "VDINR_MSAOnVCU_flg"
  Cast620/1 -> Bus1/225  "VDINR_MSAOnVCUValid_flg"
  Cast621/1 -> Bus1/240  "VDINR_DefMaxACCSetSpeed_kph"
  Cast622/1 -> Bus1/241  "VDINR_DefMaxACCSetSpeedValid_flg"
  Cast184/1 -> Bus1/36  "VDINR_OBDWarnCycAchiv_flg"
  Cast702/1 -> Bus1/37  "VDINR_OBDWarnCycAchivValid_flg"
  Cast703/1 -> Bus1/38  "VDINR_OBDDriveCycAchiv_flg"
  Cast715/1 -> Bus1/39  "VDINR_OBDDriveCycAchivValid_flg"
  Cast397/1 -> Bus1/48  "VDINR_TqConvClutchSt_enum"
  Cast398/1 -> Bus1/49  "VDINR_TqConvClutchStValid_flg"
  Cast442/1 -> Bus1/50  "VDINR_TCMMILReq_flg"
  Cast444/1 -> Bus1/51  "VDINR_TCMMILReqValid_flg"
  Cast445/1 -> Bus1/52  "VDINR_TCMWinterMode_flg"
  Cast463/1 -> Bus1/53  "VDINR_TCMWinterModeValid_flg"
  Cast464/1 -> Bus1/54  "VDINR_TCMPowerMode_flg"
  Cast489/1 -> Bus1/55  "VDINR_TCMPowerModeValid_flg"
  Cast573/1 -> Bus1/150  "VDINR_EPSLKAStatus_enum"
  Cast595/1 -> Bus1/151  "VDINR_EPSLKAStatusValid_flg"
  Cast421/1 -> Bus1/152  "VDINR_EPSLFCStatus_enum"
  Cast422/1 -> Bus1/153  "VDINR_EPSLFCStatusValid_flg"
  Cast423/1 -> Bus1/154  "VDINR_EPSADASAbReason_enum"
  Cast424/1 -> Bus1/155  "VDINR_EPSADASAbReasonValid_flg"
  Cast490/1 -> Bus1/170  "VDINR_RearFogSwOn_flg"
  Cast623/1 -> Bus1/171  "VDINR_RearFogSwOnValid_flg"
  Cast624/1 -> Bus1/172  "VDINR_HighBeamSwOn_flg"
  Cast625/1 -> Bus1/173  "VDINR_HighBeamSwOnValid_flg"
  Cast510/1 -> Bus1/202  "VDINR_TCMGearPosnReqAllow_enum"
  Cast511/1 -> Bus1/203  "VDINR_TCMGearPosnReqAllowValid_flg"
  Cast530/1 -> Bus1/204  "VDINR_MSAStatus_enum"
  Cast531/1 -> Bus1/205  "VDINR_MSAStatusValid_flg"
  Cast626/1 -> Bus1/206  "VDINR_HybridLimpHome_flg"
  Cast627/1 -> Bus1/207  "VDINR_HybridLimpHomeValid_flg"
  Cast629/1 -> Bus1/210  "VDINR_ACCOnVCU_flg"
  Cast630/1 -> Bus1/211  "VDINR_ACCOnVCUValid_flg"
  Cast631/1 -> Bus1/212  "VDINR_ACCResSpdIncVCU_flg"
  Cast632/1 -> Bus1/213  "VDINR_ACCResSpdIncVCUValid_flg"
  Cast633/1 -> Bus1/214  "VDINR_ACCSetSpdDecVCU_flg"
  Cast634/1 -> Bus1/215  "VDINR_ACCSetSpdDecVCUValid_flg"
  Cast635/1 -> Bus1/216  "VDINR_ACCDistVCU_flg"
  Cast636/1 -> Bus1/217  "VDINR_ACCDistVCUValid_flg"
  Cast534/1 -> Bus1/308  "VDINR_ViewRangeEndR_m"
  Cast535/1 -> Bus1/309  "VDINR_ViewRangeEndRValid_flg"
  Cast536/1 -> Bus1/306  "VDINR_ViewRangeEndL_m"
  Cast537/1 -> Bus1/307  "VDINR_ViewRangeEndLValid_flg"
  Cast538/1 -> Bus1/354  "VDINR_CamNofObjects_num"
  Cast540/1 -> Bus1/355  "VDINR_CamNofObjectsValid_flg"
  Cast592/1 -> Bus1/356  "VDINR_CamGoDecision_enum"
  Cast593/1 -> Bus1/357  "VDINR_CamGoDecisionValid_flg"
  Cast594/1 -> Bus1/358  "VDINR_CloseCarDetected_flg"
  Cast596/1 -> Bus1/359  "VDINR_CloseCarDetectedValid_flg"
  Cast637/1 -> Bus1/360  "VDINR_RightCarCutIn_flg"
  Cast638/1 -> Bus1/361  "VDINR_RightCarCutInValid_flg"
  Cast640/1 -> Bus1/362  "VDINR_LeftCarCutIn_flg"
  Cast641/1 -> Bus1/363  "VDINR_LeftCarCutInValid_flg"
  Cast642/1 -> Bus1/364  "VDINR_CamFSImpairedVD_flg"
  Cast643/1 -> Bus1/365  "VDINR_CamFSImpairedVDValid_flg"
  Cast644/1 -> Bus1/366  "VDINR_CamFSLowSun_flg"
  Cast645/1 -> Bus1/367  "VDINR_CamFSLowSunValid_flg"
  Cast646/1 -> Bus1/368  "VDINR_CamFSBlurImage_flg"
  Cast647/1 -> Bus1/369  "VDINR_CamFSBlurImageValid_flg"
  Cast648/1 -> Bus1/370  "VDINR_CamFSSmearImage_flg"
  Cast649/1 -> Bus1/371  "VDINR_CamFSSmearImageValid_flg"
  Cast651/1 -> Bus1/372  "VDINR_CamFSPartialBlockage_flg"
  Cast652/1 -> Bus1/373  "VDINR_CamFSPartialBlockageValid_flg"
  Cast653/1 -> Bus1/374  "VDINR_CamFSFullBlockage_flg"
  Cast654/1 -> Bus1/375  "VDINR_CamFSFullBlockageValid_flg"
  Cast655/1 -> Bus1/376  "VDINR_CamFSSplashes_flg"
  Cast656/1 -> Bus1/377  "VDINR_CamFSSplashesValid_flg"
  Cast657/1 -> Bus1/378  "VDINR_CamFSOutofCal_flg"
  Cast658/1 -> Bus1/379  "VDINR_CamFSOutofCalValid_flg"
  Cast659/1 -> Bus1/380  "VDINR_CamFSCalMisalign_flg"
  Cast660/1 -> Bus1/381  "VDINR_CamFSCalMisalignValid_flg"
  Cast662/1 -> Bus1/382  "VDINR_CamFSSmearedspots_flg"
  Cast663/1 -> Bus1/383  "VDINR_CamFSSmearedspotsValid_flg"
  Cast664/1 -> Bus1/384  "VDINR_CamFSSpotHalosFrozen_flg"
  Cast665/1 -> Bus1/385  "VDINR_CamFSSpotHalosFrozenValid_flg"
  Cast666/1 -> Bus1/386  "VDINR_CamFSFoggySpots_flg"
  Cast667/1 -> Bus1/387  "VDINR_CamFSFoggySpotsValid_flg"
  Cast668/1 -> Bus1/388  "VDINR_CamFSSunRay_flg"
  Cast669/1 -> Bus1/389  "VDINR_CamFSSunRayValid_flg"
  Cast670/1 -> Bus1/452  "VDINR_CSWCANValid_flg"
  Cast671/1 -> Bus1/464  "VDINR_CSWCANAlive_flg"
  Cast733/1 -> Bus1/60, [VDINR_TurnSignalSwL_flg]  "VDINR_TurnSignalSwL_flg"
  Cast734/1 -> Bus1/62, [VDINR_TurnSignalSwR_flg]  "VDINR_TurnSignalSwR_flg"
  Cast682/1 -> Bus1/274, [VDINR_LaneC0LRaw_m]  "VDINR_LaneC0LRaw_m"
  Cast683/1 -> Bus1/276, [VDINR_LaneC1LRaw_rad]  "VDINR_LaneC1LRaw_rad"
  Cast685/1 -> Bus1/278, [VDINR_LaneC2LRaw_rat]  "VDINR_LaneC2LRaw_rat"
  Cast686/1 -> Bus1/280, [VDINR_LaneC3LRaw_rat]  "VDINR_LaneC3LRaw_rat"
  Cast687/1 -> Bus1/282, [VDINR_LaneC0RRaw_m]  "VDINR_LaneC0RRaw_m"
  Cast688/1 -> Bus1/284, [VDINR_LaneC1RRaw_rad]  "VDINR_LaneC1RRaw_rad"
  Cast689/1 -> Bus1/286, [VDINR_LaneC2RRaw_rat]  "VDINR_LaneC2RRaw_rat"
  Cast690/1 -> Bus1/288, [VDINR_LaneC3RRaw_rat]  "VDINR_LaneC3RRaw_rat"
  Cast707/1 -> Bus1/434, [VDINR_LaneC0LKalF_m]  "VDINR_LaneC0LKalF_m"
  Cast708/1 -> Bus1/435, [VDINR_LaneC1LKalF_rad]  "VDINR_LaneC1LKalF_rad"
  Cast709/1 -> Bus1/436, [VDINR_LaneC2LKalF_rat]  "VDINR_LaneC2LKalF_rat"
  Cast710/1 -> Bus1/437, [VDINR_LaneC3LKalF_rat]  "VDINR_LaneC3LKalF_rat"
  Cast711/1 -> Bus1/438, [VDINR_LaneC0RKalF_m]  "VDINR_LaneC0RKalF_m"
  Cast712/1 -> Bus1/439, [VDINR_LaneC1RKalF_rad]  "VDINR_LaneC1RKalF_rad"
  Cast713/1 -> Bus1/440, [VDINR_LaneC2RKalF_rat]  "VDINR_LaneC2RKalF_rat"
  Cast714/1 -> Bus1/441, [VDINR_LaneC3RKalF_rat]  "VDINR_LaneC3RKalF_rat"
  Bus Selector/1 -> Cast461/1  "<VINP_IgnitionVolt_V>"
  Bus Selector/4 -> Cast609/1  "<VINP_BatteryVoltValid_flg>"
  Bus Selector/5 -> Cast706/1  "<VINP_AppTime_ms>"
  Bus Selector/3 -> Cast608/1  "<VINP_BatteryVolt_V>"
  Bus Selector/2 -> Cast572/1  "<VINP_IgnitionVoltValid_flg>"
  Bus Selector/10 -> Cast362/1  "<VINP_VREF1Fault_enum>"
  Bus Selector/6 -> Cast358/1  "<VINP_ADCFault_enum>"
  Bus Selector/7 -> Cast717/1  "<VINP_EEPROMFault_enum>"
  Bus Selector/8 -> Cast728/1  "<VINP_RAMFault_enum>"
  Bus Selector/9 -> Cast185/1  "<VINP_ROMFault_enum>"
  Bus Selector/13 -> Cast679/1  "<VINP_AccelPedalPosnValid_flg>"
  Bus Selector/16 -> Cast388/1  "<VINP_EngSpd_erpm>"
  Bus Selector/17 -> Cast389/1  "<VINP_EngSpdValid_flg>"
  Bus Selector/15 -> Cast387/1  "<VINP_EffAccelPedalPosnValid_flg>"
  Bus Selector/11 -> Cast373/1  "<VINP_VREF2Fault_enum>"
  Bus Selector/12 -> Cast677/1  "<VINP_AccelPedalPosn_pct>"
  Bus Selector/14 -> Cast386/1  "<VINP_EffAccelPedalPosn_pct>"
  Bus Selector/21 -> Cast448/1  "<VINP_EngTqIndicatedValid_flg>"
  Bus Selector/22 -> Cast449/1  "<VINP_EngTqIndicatedCOR_Nm>"
  Bus Selector/23 -> Cast451/1  "<VINP_EngTqIndicatedCORValid_flg>"
  Bus Selector/24 -> Cast392/1  "<VINP_EngTqMax_Nm>"
  Bus Selector/20 -> Cast447/1  "<VINP_EngTqIndicated_Nm>"
  Bus Selector/19 -> Cast391/1  "<VINP_EngTqFrictionValid_flg>"
  Bus Selector/18 -> Cast390/1  "<VINP_EngTqFriction_Nm>"
  Bus Selector/30 -> Cast455/1  "<VINP_EMSHybridOpState_enum>"
  Bus Selector/31 -> Cast456/1  "<VINP_EMSHybridOpStateValid_flg>"
  Bus Selector/26 -> Cast394/1  "<VINP_EngTqMin_Nm>"
  Bus Selector/29 -> Cast454/1  "<VINP_EngTqUnCORFaultValid_flg>"
  Bus Selector/25 -> Cast393/1  "<VINP_EngTqMaxValid_flg>"
  Bus Selector/27 -> Cast396/1  "<VINP_EngTqMinValid_flg>"
  Bus Selector/28 -> Cast452/1  "<VINP_EngTqUnCORFault_flg>"
  Bus Selector/33 -> Cast458/1  "<VINP_EMSOpStateValid_flg>"
  Bus Selector/32 -> Cast457/1  "<VINP_EMSOpState_enum>"
  Bus Selector/34 -> Cast459/1  "<VINP_EngHoodOpen_flg>"
  Bus Selector/38 -> Cast703/1  "<VINP_OBDDriveCycAchiv_flg>"
  Bus Selector/35 -> Cast460/1  "<VINP_EngHoodOpenValid_flg>"
  Bus Selector/37 -> Cast702/1  "<VINP_OBDWarnCycAchivValid_flg>"
  Bus Selector/36 -> Cast184/1  "<VINP_OBDWarnCycAchiv_flg>"
  Bus Selector/44 -> Cast467/1  "<VINP_TMTurbineSpd_rpm>"
  Bus Selector/41 -> Cast443/1  "<VINP_ShifterPosnValid_flg>"
  Bus Selector/42 -> Cast465/1  "<VINP_NowGearPosn_enum>"
  Bus Selector/39 -> Cast715/1  "<VINP_OBDDriveCycAchivValid_flg>"
  Bus Selector/40 -> Cast441/1  "<VINP_ShifterPosn_enum>"
  Bus Selector/43 -> Cast466/1  "<VINP_NowGearPosnValid_flg>"
  Bus Selector/47 -> Cast470/1  "<VINP_TCMFaultStatusValid_flg>"
  Bus Selector/45 -> Cast468/1  "<VINP_TMTurbineSpdValid_flg>"
  Bus Selector/46 -> Cast469/1  "<VINP_TCMFaultStatus_enum>"
  Bus Selector/49 -> Cast398/1  "<VINP_TqConvClutchStValid_flg>"
  Bus Selector/52 -> Cast445/1  "<VINP_TCMWinterMode_flg>"
  Bus Selector/48 -> Cast397/1  "<VINP_TqConvClutchSt_enum>"
  Bus Selector/54 -> Cast464/1  "<VINP_TCMPowerMode_flg>"
  Bus Selector/56 -> Cast471/1  "<VINP_DriverMode_enum>"
  Bus Selector/50 -> Cast442/1  "<VINP_TCMMILReq_flg>"
  Bus Selector/55 -> Cast489/1  "<VINP_TCMPowerModeValid_flg>"
  Bus Selector/51 -> Cast444/1  "<VINP_TCMMILReqValid_flg>"
  Bus Selector/57 -> Cast472/1  "<VINP_DriverModeValid_flg>"
  Bus Selector/53 -> Cast463/1  "<VINP_TCMWinterModeValid_flg>"
  Bus Selector/61 -> Cast475/1  "<VINP_TurnSignalSwLValid_flg>"
  Bus Selector/60 -> Cast733/1  "<VINP_TurnSignalSwL_flg>"
  Bus Selector/59 -> Cast453/1  "<VINP_KeySwitchStatusValid_flg>"
  Bus Selector/58 -> Cast732/1  "<VINP_KeySwitchStatus_enum>"
  Bus Selector/62 -> Cast734/1  "<VINP_TurnSignalSwR_flg>"
  Bus Selector/63 -> Cast476/1  "<VINP_TurnSignalSwRValid_flg>"
  Bus Selector/64 -> Cast474/1  "<VINP_HazardLightSw_flg>"
  Bus Selector/65 -> Cast477/1  "<VINP_HazardLightSwValid_flg>"
  Bus Selector/66 -> Cast492/1  "<VINP_DriverDoorOpen_flg>"
  Bus Selector/67 -> Cast493/1  "<VINP_DriverDoorOpenValid_flg>"
  Bus Selector/68 -> Cast494/1  "<VINP_PassengerDoorOpen_flg>"
  Bus Selector/69 -> Cast496/1  "<VINP_PassengerDoorOpenValid_flg>"
  Bus Selector/70 -> Cast497/1  "<VINP_LRDoorOpen_flg>"
  Bus Selector/71 -> Cast498/1  "<VINP_LRDoorOpenValid_flg>"
  Bus Selector/72 -> Cast673/1  "<VINP_RRDoorOpen_flg>"
  Bus Selector/73 -> Cast684/1  "<VINP_RRDoorOpenValid_flg>"
  Bus Selector/74 -> Cast384/1  "<VINP_TailGateOpen_flg>"
  Bus Selector/75 -> Cast395/1  "<VINP_TailGateOpenValid_flg>"
  Bus Selector/76 -> Cast406/1  "<VINP_AnyDoorOpen_flg>"
  Bus Selector/77 -> Cast417/1  "<VINP_AnyDoorOpenValid_flg>"
  Bus Selector/78 -> Cast428/1  "<VINP_VehCrashed_flg>"
  Bus Selector/79 -> Cast439/1  "<VINP_VehCrashedValid_flg>"
  Bus Selector/80 -> Cast716/1  "<VINP_ABSActive_flg>"
  Bus Selector/81 -> Cast478/1  "<VINP_ABSActiveValid_flg>"
  Bus Selector/82 -> Cast718/1  "<VINP_ABSFault_flg>"
  Bus Selector/83 -> Cast479/1  "<VINP_ABSFaultValid_flg>"
  Bus Selector/84 -> Cast721/1  "<VINP_EBDFault_flg>"
  Bus Selector/85 -> Cast480/1  "<VINP_EBDFaultValid_flg>"
  Bus Selector/86 -> Cast722/1  "<VINP_ESCActive_flg>"
  Bus Selector/87 -> Cast481/1  "<VINP_ESCActiveValid_flg>"
  Bus Selector/88 -> Cast723/1  "<VINP_ESCFault_flg>"
  Bus Selector/89 -> Cast482/1  "<VINP_ESCFaultValid_flg>"
  Bus Selector/90 -> Cast724/1  "<VINP_TCSActive_flg>"
  Bus Selector/91 -> Cast483/1  "<VINP_TCSActiveValid_flg>"
  Bus Selector/92 -> Cast725/1  "<VINP_TCSEnabled_flg>"
  Bus Selector/93 -> Cast485/1  "<VINP_TCSEnabledValid_flg>"
  Bus Selector/94 -> Cast726/1  "<VINP_TCSFault_flg>"
  Bus Selector/95 -> Cast486/1  "<VINP_TCSFaultValid_flg>"
  Bus Selector/96 -> Cast450/1  "<VINP_HSAActive_flg>"
  Bus Selector/97 -> Cast462/1  "<VINP_HSAActiveValid_flg>"
  Bus Selector/98 -> Cast473/1  "<VINP_HSAFault_flg>"
  Bus Selector/99 -> Cast484/1  "<VINP_HSAFaultValid_flg>"
  Bus Selector/100 -> Cast719/1  "<VINP_BrkLampOn_flg>"
  Bus Selector/101 -> Cast720/1  "<VINP_BrkLampOnValid_flg>"
  Bus Selector/102 -> Cast727/1  "<VINP_VehSpd_kph>"
  Bus Selector/103 -> Cast729/1  "<VINP_VehSpdValid_flg>"
  Bus Selector/104 -> Cast488/1  "<VINP_YawRate_degps>"
  Bus Selector/105 -> Cast731/1  "<VINP_YawRateValid_flg>"
  Bus Selector/106 -> Cast402/1  "<VINP_LatAccel_G>"
  Bus Selector/107 -> Cast401/1  "<VINP_LatAccelValid_flg>"
  Bus Selector/108 -> Cast404/1  "<VINP_LongAccel_G>"
  Bus Selector/109 -> Cast403/1  "<VINP_LongAccelValid_flg>"
  Bus Selector/110 -> Cast407/1  "<VINP_MCPressure_bar>"
  Bus Selector/111 -> Cast405/1  "<VINP_MCPressureValid_flg>"
  Bus Selector/112 -> Cast506/1  "<VINP_SurfaceGrade_deg>"
  Bus Selector/113 -> Cast495/1  "<VINP_SurfaceGradeValid_flg>"
  Bus Selector/114 -> Cast528/1  "<VINP_BrakBoosterPres_kPa>"
  Bus Selector/115 -> Cast517/1  "<VINP_BrakBoosterPresValid_flg>"
  Bus Selector/116 -> Cast539/1  "<VINP_LowBrakBoosterPres_flg>"
  Bus Selector/117 -> Cast550/1  "<VINP_LowBrakBoosterPresValid_flg>"
  Bus Selector/118 -> Cast628/1  "<VINP_LFWheelSpeed_kph>"
  Bus Selector/119 -> Cast617/1  "<VINP_LFWheelSpeedValid_flg>"
  Bus Selector/120 -> Cast650/1  "<VINP_LRWheelSpeed_kph>"
  Bus Selector/121 -> Cast639/1  "<VINP_LRWheelSpeedValid_flg>"
  Bus Selector/122 -> Cast672/1  "<VINP_RFWheelSpeed_kph>"
  Bus Selector/123 -> Cast661/1  "<VINP_RFWheelSpeedValid_flg>"
  Bus Selector/124 -> Cast675/1  "<VINP_RRWheelSpeed_kph>"
  Bus Selector/125 -> Cast674/1  "<VINP_RRWheelSpeedValid_flg>"
  Bus Selector/126 -> Cast487/1  "<VINP_SteerAngle_deg>"
  Bus Selector/127 -> Cast730/1  "<VINP_SteerAngleValid_flg>"
  Bus Selector/128 -> Cast610/1  "<VINP_SteerSpeed_degps>"
  Bus Selector/129 -> Cast611/1  "<VINP_SteerSpeedValid_flg>"
  Bus Selector/130 -> Cast678/1  "<VINP_RelSteerAngle_deg>"
  Bus Selector/131 -> Cast676/1  "<VINP_RelSteerAngleValid_flg>"
  Bus Selector/132 -> Cast399/1  "<VINP_SteerTorque_Nm>"
  Bus Selector/133 -> Cast400/1  "<VINP_SteerTorqueValid_flg>"
  Bus Selector/134 -> Cast446/1  "<VINP_EPSElectPWR_A>"
  Bus Selector/135 -> Cast491/1  "<VINP_EPSElectPWRValid_flg>"
  Bus Selector/136 -> Cast408/1  "<VINP_EPSFailed_flg>"
  Bus Selector/137 -> Cast409/1  "<VINP_EPSFailedValid_flg>"
  Bus Selector/138 -> Cast411/1  "<VINP_AckCurStrAngReq_deg>"
  Bus Selector/139 -> Cast410/1  "<VINP_AckCurStrAngReqValid_flg>"
  Bus Selector/140 -> Cast412/1  "<VINP_AckCurStrAngReqApplable_flg>"
  Bus Selector/141 -> Cast413/1  "<VINP_AckCurStrAngReqApplableValid_flg>"
  Bus Selector/142 -> Cast415/1  "<VINP_AckCurStrTqReq_Nm>"
  Bus Selector/143 -> Cast414/1  "<VINP_AckCurStrTqReqValid_flg>"
  Bus Selector/144 -> Cast416/1  "<VINP_AckCurStrTqReqApplable_flg>"
  Bus Selector/145 -> Cast418/1  "<VINP_AckCurStrTqReqApplableValid_flg>"
  Bus Selector/146 -> Cast420/1  "<VINP_EPSBattVolt_V>"
  Bus Selector/147 -> Cast419/1  "<VINP_EPSBattVoltValid_flg>"
  Bus Selector/148 -> Cast612/1  "<VINP_EPASMILReq_flg>"
  Bus Selector/149 -> Cast613/1  "<VINP_EPASMILReqValid_flg>"
  Bus Selector/150 -> Cast573/1  "<VINP_EPSLKAStatus_enum>"
  Bus Selector/151 -> Cast595/1  "<VINP_EPSLKAStatusValid_flg>"
  Bus Selector/152 -> Cast421/1  "<VINP_EPSLFCStatus_enum>"
  Bus Selector/153 -> Cast422/1  "<VINP_EPSLFCStatusValid_flg>"
  Bus Selector/154 -> Cast423/1  "<VINP_EPSADASAbReason_enum>"
  Bus Selector/155 -> Cast424/1  "<VINP_EPSADASAbReasonValid_flg>"
  Bus Selector/156 -> Cast426/1  "<VINP_OdoMeter_km>"
  Bus Selector/157 -> Cast425/1  "<VINP_OdoMeterValid_flg>"
  Bus Selector/158 -> Cast427/1  "<VINP_LowBrakeFluid_flg>"
  Bus Selector/159 -> Cast429/1  "<VINP_LowBrakeFluidValid_flg>"
  Bus Selector/160 -> Cast430/1  "<VINP_ParkBrakeOn_flg>"
  Bus Selector/161 -> Cast431/1  "<VINP_ParkBrakeOnValid_flg>"
  Bus Selector/162 -> Cast432/1  "<VINP_SeatBeltNOTFasten_flg>"
  Bus Selector/163 -> Cast433/1  "<VINP_SeatBeltNOTFastenValid_flg>"
  Bus Selector/164 -> Cast435/1  "<VINP_MeterVehSpd_kph>"
  Bus Selector/165 -> Cast434/1  "<VINP_MeterVehSpdValid_flg>"
  Bus Selector/166 -> Cast437/1  "<VINP_OutsideTemp_degC>"
  Bus Selector/167 -> Cast436/1  "<VINP_OutsideTempValid_flg>"
  Bus Selector/168 -> Cast438/1  "<VINP_ParkBrakeBindSta_enum>"
  Bus Selector/169 -> Cast440/1  "<VINP_ParkBrakeBindStaValid_flg>"
  Bus Selector/170 -> Cast490/1  "<VINP_RearFogSwOn_flg>"
  Bus Selector/171 -> Cast623/1  "<VINP_RearFogSwOnValid_flg>"
  Bus Selector/172 -> Cast624/1  "<VINP_HighBeamSwOn_flg>"
  Bus Selector/173 -> Cast625/1  "<VINP_HighBeamSwOnValid_flg>"
  Bus Selector/174 -> Cast499/1  "<VINP_AckCurBrakDecReq_mps2>"
  Bus Selector/175 -> Cast500/1  "<VINP_AckCurBrakDecReqValid_flg>"
  Bus Selector/176 -> Cast501/1  "<VINP_AckCurBrakDecReqApplable_flg>"
  Bus Selector/177 -> Cast502/1  "<VINP_AckCurBrakDecReqApplableValid_flg>"
  Bus Selector/178 -> Cast503/1  "<VINP_AckCurPTTqReq_Nm>"
  Bus Selector/179 -> Cast504/1  "<VINP_AckCurPTTqReqValid_flg>"
  Bus Selector/180 -> Cast505/1  "<VINP_AckCurPTTqReqApplable_flg>"
  Bus Selector/181 -> Cast507/1  "<VINP_AckCurPTTqReqApplableValid_flg>"
  Bus Selector/182 -> Cast508/1  "<VINP_AckCurVehDec_mps2>"
  Bus Selector/183 -> Cast509/1  "<VINP_AckCurVehDecValid_flg>"
  Bus Selector/184 -> Cast512/1  "<VINP_DeceContManag_flg>"
  Bus Selector/185 -> Cast513/1  "<VINP_DeceContManagValid_flg>"
  Bus Selector/187 -> Cast515/1  "<VINP_DriverBrakPedalOnValid_flg>"
  Bus Selector/188 -> Cast516/1  "<VINP_ECMExtnTqAvailable_flg>"
  Bus Selector/189 -> Cast518/1  "<VINP_ECMExtnTqAvailableValid_flg>"
  Bus Selector/190 -> Cast519/1  "<VINP_ECMTqSource_enum>"
  Bus Selector/191 -> Cast520/1  "<VINP_ECMTqSourceValid_flg>"
  Bus Selector/192 -> Cast521/1  "<VINP_ESCBrakeStatus_enum>"
  Bus Selector/193 -> Cast522/1  "<VINP_ESCBrakeStatusValid_flg>"
  Bus Selector/194 -> Cast523/1  "<VINP_ESCExtnBrkAvailable_flg>"
  Bus Selector/195 -> Cast524/1  "<VINP_ESCExtnBrkAvailableValid_flg>"
  Bus Selector/196 -> Cast525/1  "<VINP_ESCBattVolt_V>"
  Bus Selector/197 -> Cast526/1  "<VINP_ESCBattVoltValid_flg>"
  Bus Selector/198 -> Cast527/1  "<VINP_HWAccelPedalPosn_pct>"
  Bus Selector/199 -> Cast529/1  "<VINP_HWAccelPedalPosnValid_flg>"
  Bus Selector/200 -> Cast614/1  "<VINP_CurDriverTqReq_Nm>"
  Bus Selector/201 -> Cast615/1  "<VINP_CurDriverTqReqValid_flg>"
  Bus Selector/202 -> Cast510/1  "<VINP_TCMGearPosnReqAllow_enum>"
  Bus Selector/203 -> Cast511/1  "<VINP_TCMGearPosnReqAllowValid_flg>"
  Bus Selector/204 -> Cast530/1  "<VINP_MSAStatus_enum>"
  Bus Selector/205 -> Cast531/1  "<VINP_MSAStatusValid_flg>"
  Bus Selector/206 -> Cast626/1  "<VINP_HybridLimpHome_flg>"
  Bus Selector/207 -> Cast627/1  "<VINP_HybridLimpHomeValid_flg>"
  Bus Selector/208 -> Cast532/1  "<VINP_HCUMILReq_flg>"
  Bus Selector/209 -> Cast533/1  "<VINP_HCUMILReqValid_flg>"
  Bus Selector/210 -> Cast629/1  "<VINP_ACCOnVCU_flg>"
  Bus Selector/211 -> Cast630/1  "<VINP_ACCOnVCUValid_flg>"
  Bus Selector/212 -> Cast631/1  "<VINP_ACCResSpdIncVCU_flg>"
  Bus Selector/213 -> Cast632/1  "<VINP_ACCResSpdIncVCUValid_flg>"
  Bus Selector/214 -> Cast633/1  "<VINP_ACCSetSpdDecVCU_flg>"
  Bus Selector/215 -> Cast634/1  "<VINP_ACCSetSpdDecVCUValid_flg>"
  Bus Selector/216 -> Cast635/1  "<VINP_ACCDistVCU_flg>"
  Bus Selector/217 -> Cast636/1  "<VINP_ACCDistVCUValid_flg>"
  Bus Selector/218 -> Cast541/1  "<VINP_ACCTimeGapIncVCU_flg>"
  Bus Selector/219 -> Cast542/1  "<VINP_ACCTimeGapIncVCUValid_flg>"
  Bus Selector/220 -> Cast543/1  "<VINP_ACCTimeGapDecVCU_flg>"
  Bus Selector/221 -> Cast544/1  "<VINP_ACCTimeGapDecVCUValid_flg>"
  Bus Selector/222 -> Cast545/1  "<VINP_LFCOnVCU_flg>"
  Bus Selector/223 -> Cast546/1  "<VINP_LFCOnVCUValid_flg>"
  Bus Selector/224 -> Cast619/1  "<VINP_MSAOnVCU_flg>"
  Bus Selector/225 -> Cast620/1  "<VINP_MSAOnVCUValid_flg>"
  Bus Selector/226 -> Cast547/1  "<VINP_AEBEnableH_flg>"
  Bus Selector/227 -> Cast548/1  "<VINP_AEBEnableHValid_flg>"
  Bus Selector/228 -> Cast549/1  "<VINP_FCWEnableH_flg>"
  Bus Selector/229 -> Cast551/1  "<VINP_FCWEnableHValid_flg>"
  Bus Selector/230 -> Cast552/1  "<VINP_CSCEnableH_flg>"
  Bus Selector/231 -> Cast553/1  "<VINP_CSCEnableHValid_flg>"
  Bus Selector/232 -> Cast554/1  "<VINP_LKAEnableH_flg>"
  Bus Selector/233 -> Cast555/1  "<VINP_LKAEnableHValid_flg>"
  Bus Selector/234 -> Cast556/1  "<VINP_MAPAEnableH_flg>"
  Bus Selector/235 -> Cast557/1  "<VINP_MAPAEnableHValid_flg>"
  Bus Selector/236 -> Cast558/1  "<VINP_LCSEnableH_flg>"
  Bus Selector/237 -> Cast559/1  "<VINP_LCSEnableHValid_flg>"
  Bus Selector/238 -> Cast616/1  "<VINP_FCWWarningModeH_enum>"
  Bus Selector/239 -> Cast618/1  "<VINP_FCWWarningModeHValid_flg>"
  Bus Selector/240 -> Cast621/1  "<VINP_DefMaxACCSetSpeed_kph>"
  Bus Selector/241 -> Cast622/1  "<VINP_DefMaxACCSetSpeedValid_flg>"
  Bus Selector/242 -> Cast560/1  "<VINP_LFCPilotOnH_flg>"
  Bus Selector/243 -> Cast562/1  "<VINP_LFCPilotOnHValid_flg>"
  Bus Selector/244 -> Cast563/1  "<VINP_LFCPilotCancelH_flg>"
  Bus Selector/245 -> Cast564/1  "<VINP_LFCPilotCancelHValid_flg>"
  Bus Selector/246 -> Cast565/1  "<VINP_ACCOnH_flg>"
  Bus Selector/247 -> Cast566/1  "<VINP_ACCOnHValid_flg>"
  Bus Selector/248 -> Cast567/1  "<VINP_ACCCancelH_flg>"
  Bus Selector/249 -> Cast568/1  "<VINP_ACCCancelHValid_flg>"
  Bus Selector/250 -> Cast569/1  "<VINP_ACCResSpdIncH_flg>"
  Bus Selector/251 -> Cast570/1  "<VINP_ACCResSpdIncHValid_flg>"
  Bus Selector/252 -> Cast571/1  "<VINP_ACCSetSpdDecH_flg>"
  Bus Selector/253 -> Cast574/1  "<VINP_ACCSetSpdDecHValid_flg>"
  Bus Selector/254 -> Cast575/1  "<VINP_ACCSpdIncH_flg>"
  Bus Selector/255 -> Cast576/1  "<VINP_ACCSpdIncHValid_flg>"
  Bus Selector/256 -> Cast577/1  "<VINP_ACCSpdDecH_flg>"
  Bus Selector/257 -> Cast578/1  "<VINP_ACCSpdDecHValid_flg>"
  Bus Selector/258 -> Cast579/1  "<VINP_ACCTimeGapIncH_flg>"
  Bus Selector/259 -> Cast580/1  "<VINP_ACCTimeGapIncHValid_flg>"
  Bus Selector/260 -> Cast581/1  "<VINP_ACCTimeGapDecH_flg>"
  Bus Selector/261 -> Cast582/1  "<VINP_ACCTimeGapDecHValid_flg>"
  Bus Selector/262 -> Cast583/1  "<VINP_IGSAOnH_flg>"
  Bus Selector/263 -> Cast585/1  "<VINP_IGSAOnHValid_flg>"
  Bus Selector/264 -> Cast586/1  "<VINP_IGSAResSpdIncH_flg>"
  Bus Selector/265 -> Cast587/1  "<VINP_IGSAResSpdIncHValid_flg>"
  Bus Selector/266 -> Cast588/1  "<VINP_IGSASetSpdDecH_flg>"
  Bus Selector/267 -> Cast589/1  "<VINP_IGSASetSpdDecHValid_flg>"
  Bus Selector/268 -> Cast590/1  "<VINP_IGSASwitchModeH_flg>"
  Bus Selector/269 -> Cast591/1  "<VINP_IGSASwitchModeHValid_flg>"
  Bus Selector/270 -> Cast680/1  "<VINP_LaneQualityL_enum>"
  Bus Selector/271 -> Cast735/1  "<VINP_LaneQualityLValid_flg>"
  Bus Selector/272 -> Cast681/1  "<VINP_LaneQualityR_enum>"
  Bus Selector/273 -> Cast736/1  "<VINP_LaneQualityRValid_flg>"
  Bus Selector/274 -> Cast682/1  "<VINP_LaneC0LRaw_m>"
  Bus Selector/275 -> Cast737/1  "<VINP_LaneC0LValid_flg>"
  Bus Selector/276 -> Cast683/1  "<VINP_LaneC1LRaw_rad>"
  Bus Selector/277 -> Cast738/1  "<VINP_LaneC1LValid_flg>"
  Bus Selector/278 -> Cast685/1  "<VINP_LaneC2LRaw_rat>"
  Bus Selector/279 -> Cast224/1  "<VINP_LaneC2LValid_flg>"
  Bus Selector/280 -> Cast686/1  "<VINP_LaneC3LRaw_rat>"
  Bus Selector/281 -> Cast225/1  "<VINP_LaneC3LValid_flg>"
  Bus Selector/282 -> Cast687/1  "<VINP_LaneC0RRaw_m>"
  Bus Selector/283 -> Cast354/1  "<VINP_LaneC0RValid_flg>"
  Bus Selector/284 -> Cast688/1  "<VINP_LaneC1RRaw_rad>"
  Bus Selector/285 -> Cast355/1  "<VINP_LaneC1RValid_flg>"
  Bus Selector/286 -> Cast689/1  "<VINP_LaneC2RRaw_rat>"
  Bus Selector/287 -> Cast356/1  "<VINP_LaneC2RValid_flg>"
  Bus Selector/288 -> Cast690/1  "<VINP_LaneC3RRaw_rat>"
  Bus Selector/289 -> Cast357/1  "<VINP_LaneC3RValid_flg>"
  Bus Selector/290 -> Cast359/1  "<VINP_LaneTypeL_enum>"
  Bus Selector/291 -> Cast360/1  "<VINP_LaneTypeLValid_flg>"
  Bus Selector/292 -> Cast361/1  "<VINP_LaneTypeR_enum>"
  Bus Selector/293 -> Cast363/1  "<VINP_LaneTypeRValid_flg>"
  Bus Selector/294 -> Cast364/1  "<VINP_LaneMrkClrL_enum>"
  Bus Selector/295 -> Cast365/1  "<VINP_LaneMrkClrLValid_flg>"
  Bus Selector/296 -> Cast366/1  "<VINP_LaneMrkClrR_enum>"
  Bus Selector/297 -> Cast367/1  "<VINP_LaneMrkClrRValid_flg>"
  Bus Selector/298 -> Cast368/1  "<VINP_LaneMrkWidL_m>"
  Bus Selector/299 -> Cast369/1  "<VINP_LaneMrkWidLValid_flg>"
  Bus Selector/300 -> Cast370/1  "<VINP_LaneMrkWidR_m>"
  Bus Selector/301 -> Cast371/1  "<VINP_LaneMrkWidRValid_flg>"
  Bus Selector/302 -> Cast372/1  "<VINP_ViewRangeStartL_m>"
  Bus Selector/303 -> Cast374/1  "<VINP_ViewRangeStartLValid_flg>"
  Bus Selector/304 -> Cast375/1  "<VINP_ViewRangeStartR_m>"
  Bus Selector/305 -> Cast376/1  "<VINP_ViewRangeStartRValid_flg>"
  Bus Selector/306 -> Cast536/1  "<VINP_ViewRangeEndL_m>"
  Bus Selector/307 -> Cast537/1  "<VINP_ViewRangeEndLValid_flg>"
  Bus Selector/308 -> Cast534/1  "<VINP_ViewRangeEndR_m>"
  Bus Selector/309 -> Cast535/1  "<VINP_ViewRangeEndRValid_flg>"
  Bus Selector/310 -> Cast377/1  "<VINP_TLCL_s>"
  Bus Selector/311 -> Cast378/1  "<VINP_TLCLValid_flg>"
  Bus Selector/312 -> Cast379/1  "<VINP_TLCR_s>"
  Bus Selector/313 -> Cast380/1  "<VINP_TLCRValid_flg>"
  Bus Selector/314 -> Cast381/1  "<VINP_LaneCrosL_flg>"
  Bus Selector/315 -> Cast382/1  "<VINP_LaneCrosLValid_flg>"
  Bus Selector/316 -> Cast383/1  "<VINP_LaneCrosR_flg>"
  Bus Selector/317 -> Cast385/1  "<VINP_LaneCrosRValid_flg>"
  Bus Selector/354 -> Cast538/1  "<VINP_CamNofObjects_num>"
  Bus Selector/355 -> Cast540/1  "<VINP_CamNofObjectsValid_flg>"
  Bus Selector/356 -> Cast592/1  "<VINP_CamGoDecision_enum>"
  Bus Selector/357 -> Cast593/1  "<VINP_CamGoDecisionValid_flg>"
  Bus Selector/358 -> Cast594/1  "<VINP_CloseCarDetected_flg>"
  Bus Selector/359 -> Cast596/1  "<VINP_CloseCarDetectedValid_flg>"
  Bus Selector/360 -> Cast637/1  "<VINP_RightCarCutIn_flg>"
  Bus Selector/361 -> Cast638/1  "<VINP_RightCarCutInValid_flg>"
  Bus Selector/362 -> Cast640/1  "<VINP_LeftCarCutIn_flg>"
  Bus Selector/363 -> Cast641/1  "<VINP_LeftCarCutInValid_flg>"
  Bus Selector/364 -> Cast642/1  "<VINP_CamFSImpairedVD_flg>"
  Bus Selector/365 -> Cast643/1  "<VINP_CamFSImpairedVDValid_flg>"
  Bus Selector/366 -> Cast644/1  "<VINP_CamFSLowSun_flg>"
  Bus Selector/367 -> Cast645/1  "<VINP_CamFSLowSunValid_flg>"
  Bus Selector/368 -> Cast646/1  "<VINP_CamFSBlurImage_flg>"
  Bus Selector/369 -> Cast647/1  "<VINP_CamFSBlurImageValid_flg>"
  Bus Selector/370 -> Cast648/1  "<VINP_CamFSSmearImage_flg>"
  Bus Selector/371 -> Cast649/1  "<VINP_CamFSSmearImageValid_flg>"
  Bus Selector/372 -> Cast651/1  "<VINP_CamFSPartialBlockage_flg>"
  Bus Selector/373 -> Cast652/1  "<VINP_CamFSPartialBlockageValid_flg>"
  Bus Selector/374 -> Cast653/1  "<VINP_CamFSFullBlockage_flg>"
  Bus Selector/375 -> Cast654/1  "<VINP_CamFSFullBlockageValid_flg>"
  Bus Selector/376 -> Cast655/1  "<VINP_CamFSSplashes_flg>"
  Bus Selector/382 -> Cast662/1  "<VINP_CamFSSmearedspots_flg>"
  Bus Selector/378 -> Cast657/1  "<VINP_CamFSOutofCal_flg>"
  Bus Selector/380 -> Cast659/1  "<VINP_CamFSCalMisalign_flg>"
  Bus Selector/377 -> Cast656/1  "<VINP_CamFSSplashesValid_flg>"
  Bus Selector/383 -> Cast663/1  "<VINP_CamFSSmearedspotsValid_flg>"
  Bus Selector/381 -> Cast660/1  "<VINP_CamFSCalMisalignValid_flg>"
  Bus Selector/385 -> Cast665/1  "<VINP_CamFSSpotHalosFrozenValid_flg>"
  Bus Selector/384 -> Cast664/1  "<VINP_CamFSSpotHalosFrozen_flg>"
  Bus Selector/379 -> Cast658/1  "<VINP_CamFSOutofCalValid_flg>"
  Bus Selector/431 -> Cast561/1  "<VINP_VehSpd_mps>"
  Bus Selector/433 -> Cast606/1  "<VINP_YawRate_radps>"
  Bus Selector/430 -> Cast695/1  "<VINP_IgnitionActive_flg>"
  Bus Selector/432 -> Cast584/1  "<VINP_SteerAngle_rad>"
  Bus Selector/388 -> Cast668/1  "<VINP_CamFSSunRay_flg>"
  Bus Selector/387 -> Cast667/1  "<VINP_CamFSFoggySpotsValid_flg>"
  Bus Selector/386 -> Cast666/1  "<VINP_CamFSFoggySpots_flg>"
  Bus Selector/389 -> Cast669/1  "<VINP_CamFSSunRayValid_flg>"
  Bus Selector/439 -> Cast712/1  "<VINP_LaneC1RKalF_rad>"
  Bus Selector/440 -> Cast713/1  "<VINP_LaneC2RKalF_rat>"
  Bus Selector/434 -> Cast707/1  "<VINP_LaneC0LKalF_m>"
  Bus Selector/436 -> Cast709/1  "<VINP_LaneC2LKalF_rat>"
  Bus Selector/435 -> Cast708/1  "<VINP_LaneC1LKalF_rad>"
  Bus Selector/438 -> Cast711/1  "<VINP_LaneC0RKalF_m>"
  Bus Selector/437 -> Cast710/1  "<VINP_LaneC3LKalF_rat>"
  Bus Selector/441 -> Cast714/1  "<VINP_LaneC3RKalF_rat>"
  Bus Selector/444 -> Cast597/1  "<VINP_ECMCANValid_flg>"
  Bus Selector/443 -> Cast704/1  "<VINP_BCMCANValid_flg>"
  Bus Selector/451 -> Cast603/1  "<VINP_HMICANValid_flg>"
  Bus Selector/449 -> Cast693/1  "<VINP_EPBCANValid_flg>"
  Bus Selector/445 -> Cast599/1  "<VINP_TCMCANValid_flg>"
  Bus Selector/448 -> Cast692/1  "<VINP_ACCANValid_flg>"
  Bus Selector/450 -> Cast694/1  "<VINP_VCUCANValid_flg>"
  Bus Selector/442 -> Cast700/1  "<VINP_ABSCANValid_flg>"
  Bus Selector/447 -> Cast691/1  "<VINP_METERCANValid_flg>"
  Bus Selector/446 -> Cast601/1  "<VINP_EPSCANValid_flg>"
  Bus Selector/460 -> Cast697/1  "<VINP_ACCANAlive_flg>"
  Bus Selector/459 -> Cast696/1  "<VINP_METERCANAlive_flg>"
  Bus Selector/453 -> Cast604/1  "<VINP_EPMCANValid_flg>"
  Bus Selector/458 -> Cast602/1  "<VINP_EPSCANAlive_flg>"
  Bus Selector/452 -> Cast670/1  "<VINP_CSWCANValid_flg>"
  Bus Selector/454 -> Cast701/1  "<VINP_ABSCANAlive_flg>"
  Bus Selector/455 -> Cast705/1  "<VINP_BCMCANAlive_flg>"
  Bus Selector/456 -> Cast598/1  "<VINP_ECMCANAlive_flg>"
  Bus Selector/457 -> Cast600/1  "<VINP_TCMCANAlive_flg>"
  Bus Selector/461 -> Cast698/1  "<VINP_EPBCANAlive_flg>"
  Bus Selector/465 -> Cast607/1  "<VINP_EPMCANAlive_flg>"
  Bus Selector/464 -> Cast671/1  "<VINP_CSWCANAlive_flg>"
  Bus Selector/463 -> Cast605/1  "<VINP_HMICANAlive_flg>"
  Bus Selector/462 -> Cast699/1  "<VINP_VCUCANAlive_flg>"
  Cast1/1 -> Bus1/466  "VDINR_CamInternalError_flg"
  Constant/1 -> Cast1/1
  Bus Selector/390 -> Cast2/1  "<VINP_CamObsID10_num>"
  Bus Selector/391 -> Cast3/1  "<VINP_CamObsIDValid10_flg>"
  Cast2/1 -> Bus1/390  "VDINR_CamObsID10_num"
  Cast3/1 -> Bus1/391  "VDINR_CamObsIDValid10_flg"
  Cast4/1 -> Bus1/392  "VDINR_CamObsPosX10_m"
  Cast5/1 -> Bus1/393  "VDINR_CamObsPosXValid10_flg"
  Bus Selector/392 -> Cast4/1  "<VINP_CamObsPosX10_m>"
  Bus Selector/393 -> Cast5/1  "<VINP_CamObsPosXValid10_flg>"
  Cast6/1 -> Bus1/394  "VDINR_CamObsPosY10_m"
  Cast7/1 -> Bus1/395  "VDINR_CamObsPosYValid10_flg"
  Bus Selector/394 -> Cast6/1  "<VINP_CamObsPosY10_m>"
  Bus Selector/395 -> Cast7/1  "<VINP_CamObsPosYValid10_flg>"
  Cast8/1 -> Bus1/396  "VDINR_CamObsVelX10_mps"
  Cast9/1 -> Bus1/397  "VDINR_CamObsVelXValid10_flg"
  Bus Selector/396 -> Cast8/1  "<VINP_CamObsVelX10_mps>"
  Bus Selector/397 -> Cast9/1  "<VINP_CamObsVelXValid10_flg>"
  Cast10/1 -> Bus1/398  "VDINR_CamObsVelY10_mps"
  Cast11/1 -> Bus1/399  "VDINR_CamObsVelYValid10_flg"
  Bus Selector/398 -> Cast10/1  "<VINP_CamObsVelY10_mps>"
  Bus Selector/399 -> Cast11/1  "<VINP_CamObsVelYValid10_flg>"
  Cast12/1 -> Bus1/400  "VDINR_CamObsAccX10_mps2"
  Cast13/1 -> Bus1/401  "VDINR_CamObsAccXValid10_flg"
  Bus Selector/400 -> Cast12/1  "<VINP_CamObsAccX10_mps2>"
  Bus Selector/401 -> Cast13/1  "<VINP_CamObsAccXValid10_flg>"
  Cast14/1 -> Bus1/402  "VDINR_CamObsAng10_deg"
  Cast15/1 -> Bus1/403  "VDINR_CamObsAngValid10_flg"
  Bus Selector/402 -> Cast14/1  "<VINP_CamObsAng10_deg>"
  Bus Selector/403 -> Cast15/1  "<VINP_CamObsAngValid10_flg>"
  Cast16/1 -> Bus1/404  "VDINR_CamObsAngRate10_degps"
  Cast17/1 -> Bus1/405  "VDINR_CamObsAngRateValid10_flg"
  Bus Selector/404 -> Cast16/1  "<VINP_CamObsAngRate10_degps>"
  Bus Selector/405 -> Cast17/1  "<VINP_CamObsAngRateValid10_flg>"
  Cast18/1 -> Bus1/406  "VDINR_CamObsLength10_m"
  Cast19/1 -> Bus1/407  "VDINR_CamObsLengthValid10_flg"
  Bus Selector/406 -> Cast18/1  "<VINP_CamObsLength10_m>"
  Bus Selector/407 -> Cast19/1  "<VINP_CamObsLengthValid10_flg>"
  Cast20/1 -> Bus1/408  "VDINR_CamObsWidth10_m"
  Cast21/1 -> Bus1/409  "VDINR_CamObsWidthValid10_flg"
  Bus Selector/408 -> Cast20/1  "<VINP_CamObsWidth10_m>"
  Bus Selector/409 -> Cast21/1  "<VINP_CamObsWidthValid10_flg>"
  Cast22/1 -> Bus1/410  "VDINR_CamObsType10_enum"
  Cast23/1 -> Bus1/411  "VDINR_CamObsTypeValid10_flg"
  Bus Selector/410 -> Cast22/1  "<VINP_CamObsType10_enum>"
  Bus Selector/411 -> Cast23/1  "<VINP_CamObsTypeValid10_flg>"
  Cast24/1 -> Bus1/412  "VDINR_CamObsStatus10_enum"
  Cast25/1 -> Bus1/413  "VDINR_CamObsStatusValid10_flg"
  Bus Selector/412 -> Cast24/1  "<VINP_CamObsStatus10_enum>"
  Bus Selector/413 -> Cast25/1  "<VINP_CamObsStatusValid10_flg>"
  Cast26/1 -> Bus1/414  "VDINR_CamObsValid10_enum"
  Cast27/1 -> Bus1/415  "VDINR_CamObsValidValid10_flg"
  Bus Selector/414 -> Cast26/1  "<VINP_CamObsValid10_enum>"
  Bus Selector/415 -> Cast27/1  "<VINP_CamObsValidValid10_flg>"
  Cast28/1 -> Bus1/416  "VDINR_CamObsMoveInO10_enum"
  Cast29/1 -> Bus1/417  "VDINR_CamObsMoveInOValid10_flg"
  Bus Selector/416 -> Cast28/1  "<VINP_CamObsMoveInO10_enum>"
  Bus Selector/417 -> Cast29/1  "<VINP_CamObsMoveInOValid10_flg>"
  Cast30/1 -> Bus1/418  "VDINR_CamObsBlinker10_enum"
  Cast31/1 -> Bus1/419  "VDINR_CamObsBlinkerValid10_flg"
  Bus Selector/418 -> Cast30/1  "<VINP_CamObsBlinker10_enum>"
  Bus Selector/419 -> Cast31/1  "<VINP_CamObsBlinkerValid10_flg>"
  Cast32/1 -> Bus1/420  "VDINR_CamObsBrakeLight10_flg"
  Cast33/1 -> Bus1/421  "VDINR_CamObsBrakeLightValid10_flg"
  Bus Selector/420 -> Cast32/1  "<VINP_CamObsBrakeLight10_flg>"
  Bus Selector/421 -> Cast33/1  "<VINP_CamObsBrakeLightValid10_flg>"
  Cast34/1 -> Bus1/422  "VDINR_CamObsAge10_cnt"
  Cast35/1 -> Bus1/423  "VDINR_CamObsAgeValid10_flg"
  Bus Selector/422 -> Cast34/1  "<VINP_CamObsAge10_cnt>"
  Bus Selector/423 -> Cast35/1  "<VINP_CamObsAgeValid10_flg>"
  Cast36/1 -> Bus1/424  "VDINR_CamObsLane10_enum"
  Cast37/1 -> Bus1/425  "VDINR_CamObsLaneValid10_flg"
  Bus Selector/424 -> Cast36/1  "<VINP_CamObsLane10_enum>"
  Bus Selector/425 -> Cast37/1  "<VINP_CamObsLaneValid10_flg>"
  Cast38/1 -> Bus1/426  "VDINR_CamObsCIPV10_flg"
  Cast39/1 -> Bus1/427  "VDINR_CamObsCIPVValid10_flg"
  Bus Selector/426 -> Cast38/1  "<VINP_CamObsCIPV10_flg>"
  Bus Selector/427 -> Cast39/1  "<VINP_CamObsCIPVValid10_flg>"
  Cast40/1 -> Bus1/428  "VDINR_CamObsReplaced10_flg"
  Cast41/1 -> Bus1/429  "VDINR_CamObsReplacedValid10_flg"
  Bus Selector/428 -> Cast40/1  "<VINP_CamObsReplaced10_flg>"
  Bus Selector/429 -> Cast41/1  "<VINP_CamObsReplacedValid10_flg>"
  Cast42/1 -> Bus1/467  "VDINR_FCWEnableO_flg"
  Constant1/1 -> Cast42/1
  Cast43/1 -> Bus1/468  "VDINR_AEBEnableO_flg"
  Constant2/1 -> Cast43/1
  Cast44/1 -> Bus1/318  "VDINR_NextLaneC0L_m"
  Cast45/1 -> Bus1/320  "VDINR_NextLaneC1L_rad"
  Cast46/1 -> Bus1/319  "VDINR_NextLaneC0LValid_flg"
  Cast47/1 -> Bus1/321  "VDINR_NextLaneC1LValid_flg"
  Cast48/1 -> Bus1/322  "VDINR_NextLaneC2L_rat"
  Cast49/1 -> Bus1/323  "VDINR_NextLaneC2LValid_flg"
  Cast50/1 -> Bus1/324  "VDINR_NextLaneC3L_rat"
  Cast51/1 -> Bus1/325  "VDINR_NextLaneC3LValid_flg"
  Cast52/1 -> Bus1/326  "VDINR_NextLaneQualityL_enum"
  Cast53/1 -> Bus1/327  "VDINR_NextLaneQualityLValid_flg"
  Cast54/1 -> Bus1/328  "VDINR_NextLaneTypeL_enum"
  Cast55/1 -> Bus1/329  "VDINR_NextLaneTypeLValid_flg"
  Cast56/1 -> Bus1/330  "VDINR_NextLaneMrkWidL_m"
  Cast57/1 -> Bus1/331  "VDINR_NextLaneMrkWidLValid_flg"
  Cast58/1 -> Bus1/332  "VDINR_NextViewRangeStartL_m"
  Cast59/1 -> Bus1/333  "VDINR_NextViewRangeStartLValid_flg"
  Cast60/1 -> Bus1/334  "VDINR_NextViewRangeEndL_m"
  Cast61/1 -> Bus1/335  "VDINR_NextViewRangeEndLValid_flg"
  Cast62/1 -> Bus1/336  "VDINR_NextLaneC0R_m"
  Cast63/1 -> Bus1/338  "VDINR_NextLaneC1R_rad"
  Cast64/1 -> Bus1/337  "VDINR_NextLaneC0RValid_flg"
  Cast65/1 -> Bus1/339  "VDINR_NextLaneC1RValid_flg"
  Cast66/1 -> Bus1/340  "VDINR_NextLaneC2R_rat"
  Cast67/1 -> Bus1/341  "VDINR_NextLaneC2RValid_flg"
  Cast68/1 -> Bus1/342  "VDINR_NextLaneC3R_rat"
  Cast69/1 -> Bus1/343  "VDINR_NextLaneC3RValid_flg"
  Cast70/1 -> Bus1/344  "VDINR_NextLaneQualityR_enum"
  Cast71/1 -> Bus1/345  "VDINR_NextLaneQualityRValid_flg"
  Cast72/1 -> Bus1/346  "VDINR_NextLaneTypeR_enum"
  Cast73/1 -> Bus1/347  "VDINR_NextLaneTypeRValid_flg"
  Cast74/1 -> Bus1/348  "VDINR_NextLaneMrkWidR_m"
  Cast75/1 -> Bus1/349  "VDINR_NextLaneMrkWidRValid_flg"
  Cast76/1 -> Bus1/350  "VDINR_NextViewRangeStartR_m"
  Cast77/1 -> Bus1/351  "VDINR_NextViewRangeStartRValid_flg"
  Cast78/1 -> Bus1/352  "VDINR_NextViewRangeEndR_m"
  Cast79/1 -> Bus1/353  "VDINR_NextViewRangeEndRValid_flg"
  Bus Selector/335 -> Cast61/1  "<VINP_NextViewRangeEndLValid_flg>"
  Bus Selector/334 -> Cast60/1  "<VINP_NextViewRangeEndL_m>"
  Bus Selector/328 -> Cast54/1  "<VINP_NextLaneTypeL_enum>"
  Bus Selector/318 -> Cast44/1  "<VINP_NextLaneC0L_m>"
  Bus Selector/321 -> Cast47/1  "<VINP_NextLaneC1LValid_flg>"
  Bus Selector/322 -> Cast48/1  "<VINP_NextLaneC2L_rat>"
  Bus Selector/327 -> Cast53/1  "<VINP_NextLaneQualityLValid_flg>"
  Bus Selector/320 -> Cast45/1  "<VINP_NextLaneC1L_rad>"
  Bus Selector/326 -> Cast52/1  "<VINP_NextLaneQualityL_enum>"
  Bus Selector/324 -> Cast50/1  "<VINP_NextLaneC3L_rat>"
  Bus Selector/330 -> Cast56/1  "<VINP_NextLaneMrkWidL_m>"
  Bus Selector/332 -> Cast58/1  "<VINP_NextViewRangeStartL_m>"
  Bus Selector/336 -> Cast62/1  "<VINP_NextLaneC0R_m>"
  Bus Selector/329 -> Cast55/1  "<VINP_NextLaneTypeLValid_flg>"
  Bus Selector/331 -> Cast57/1  "<VINP_NextLaneMrkWidLValid_flg>"
  Bus Selector/347 -> Cast73/1  "<VINP_NextLaneTypeRValid_flg>"
  Bus Selector/319 -> Cast46/1  "<VINP_NextLaneC0LValid_flg>"
  Bus Selector/348 -> Cast74/1  "<VINP_NextLaneMrkWidR_m>"
  Bus Selector/323 -> Cast49/1  "<VINP_NextLaneC2LValid_flg>"
  Bus Selector/344 -> Cast70/1  "<VINP_NextLaneQualityR_enum>"
  Bus Selector/353 -> Cast79/1  "<VINP_NextViewRangeEndRValid_flg>"
  Bus Selector/325 -> Cast51/1  "<VINP_NextLaneC3LValid_flg>"
  Bus Selector/333 -> Cast59/1  "<VINP_NextViewRangeStartLValid_flg>"
  Bus Selector/341 -> Cast67/1  "<VINP_NextLaneC2RValid_flg>"
  Bus Selector/337 -> Cast64/1  "<VINP_NextLaneC0RValid_flg>"
  Bus Selector/339 -> Cast65/1  "<VINP_NextLaneC1RValid_flg>"
  Bus Selector/338 -> Cast63/1  "<VINP_NextLaneC1R_rad>"
  Bus Selector/343 -> Cast69/1  "<VINP_NextLaneC3RValid_flg>"
  Bus Selector/345 -> Cast71/1  "<VINP_NextLaneQualityRValid_flg>"
  Bus Selector/342 -> Cast68/1  "<VINP_NextLaneC3R_rat>"
  Bus Selector/350 -> Cast76/1  "<VINP_NextViewRangeStartR_m>"
  Bus Selector/346 -> Cast72/1  "<VINP_NextLaneTypeR_enum>"
  Bus Selector/349 -> Cast75/1  "<VINP_NextLaneMrkWidRValid_flg>"
  Bus Selector/352 -> Cast78/1  "<VINP_NextViewRangeEndR_m>"
  Bus Selector/340 -> Cast66/1  "<VINP_NextLaneC2R_rat>"
  Bus Selector/351 -> Cast77/1  "<VINP_NextViewRangeStartRValid_flg>"
  [VDINR_BrkLampOn_flg] -> Terminator/1
  Bus Selector/186 -> Cast514/1  "<VINP_DriverBrakPedalOn_flg>"
